simulink model "ASM_Traffic_V2X_Complete_Model_2"  (R2019a)
(part 8 of 36)

  Angle_RL_Wheel[Toe;Camber][deg]/2 -> SignalFilter/624  "<Angle_Camber_RL_Wheel_CoorSys_V[deg]>"
  Angle_RR_Wheel[Toe;Camber][deg]/1 -> SignalFilter/625  "<Angle_Toe_RR_Wheel_CoorSys_V[deg]>"
  Angle_RR_Wheel[Toe;Camber][deg]/2 -> SignalFilter/626  "<Angle_Camber_RR_Wheel_CoorSys_V[deg]>"
  EngineTorques/1 -> SignalFilter/627  "<Const_TimeConst[s]>"
  EngineTorques/2 -> SignalFilter/628  "<Trq_Eff_Engine[Nm]>"
  EngineTorques/3 -> SignalFilter/629  "<Trq_Driver_Des[Nm]>"
  EngineTorques/4 -> SignalFilter/630  "<Trq_Fric_Engine[Nm]>"
  EngineTorques/5 -> SignalFilter/631  "<Trq_Ind_Engine[Nm]>"
  EngineTorques/6 -> SignalFilter/632  "<Trq_FullLoad_Engine[Nm]>"
  FuelConsumption/1 -> SignalFilter/633  "<mdot_Fuel[g|h]>"
  FuelConsumption/2 -> SignalFilter/634  "<b_e[g|kWh]>"
  Efficiency/1 -> SignalFilter/635  "<eta_Eff_Engine[0_1]>"
  Efficiency/2 -> SignalFilter/636  "<eta_Ind_Engine[0_1]>"
  Efficiency/3 -> SignalFilter/637  "<eta_Mechanical_Engine[0_1]>"
  CO2_Emission/1 -> SignalFilter/638  "<CO2_Emission[kg|h]>"
  CO2_Emission/2 -> SignalFilter/639  "<CO2_Emission_Total[kg]>"
  FuelConsumption/5 -> SignalFilter/640  "<Fuel_Consumption[l|h]>"
  FuelConsumption/6 -> SignalFilter/641  "<Fuel_Consumption_Total[l]>"
  ActiveTransmission/1 -> SignalFilter/642  "<Gear[]>"
  ActiveTransmission/2 -> SignalFilter/643  "<omega_In_Trm[rad|s]>"
  ActiveTransmission/3 -> SignalFilter/644  "<omega_Out_Trm[rad|s]>"
  ActiveTransmission/4 -> SignalFilter/645  "<Trq_Out_Trm[Nm]>"
  ActiveTransmission/5 -> SignalFilter/646  "<i_Trm[]>"
  ActiveTransmission/6 -> SignalFilter/647  "<Inertia_Trm[kgm2]>"
  ActiveTransmission/7 -> SignalFilter/648  "<i_unsync_Trm[]>"
  Clutch/1 -> SignalFilter/649  "<Trq_Fric_Clutch[Nm]>"
  Clutch/2 -> SignalFilter/650  "<Trq_TorsionSpring_Clutch[Nm]>"
  Clutch/3 -> SignalFilter/651  "<omega_Out_ClutchPlate[rad|s]>"
  GearBox/1 -> SignalFilter/652  "<i_unsync_Trm[]>"
  GearBox/2 -> SignalFilter/653  "<i_Trm[]>"
  GearBox/3 -> SignalFilter/654  "<Trq_Out_Trm[Nm]>"
  GearBox/4 -> SignalFilter/655  "<omega_In_Trm[rad|s]>"
  GearBox/5 -> SignalFilter/656  "<Inertia_Trm[kgm2]>"
  GearBox/6 -> SignalFilter/657  "<omega_Out_Trm[rad|s]>"
  LockUpClutch/1 -> SignalFilter/658  "<Trq_Fric_Clutch[Nm]>"
  LockUpClutch/2 -> SignalFilter/659  "<Trq_TorsionSpring_Clutch[Nm]>"
  LockUpClutch/3 -> SignalFilter/660  "<omega_Out_ClutchPlate[rad|s]>"
  GearBox1/1 -> SignalFilter/661  "<i_unsync_Trm[]>"
  GearBox1/2 -> SignalFilter/662  "<i_Trm[]>"
  GearBox1/3 -> SignalFilter/663  "<Trq_Out_Trm[Nm]>"
  GearBox1/4 -> SignalFilter/664  "<omega_In_Trm[rad|s]>"
  GearBox1/5 -> SignalFilter/665  "<Inertia_Trm[kgm2]>"
  GearBox1/6 -> SignalFilter/666  "<omega_Out_Trm[rad|s]>"
  TorqueConverter/1 -> SignalFilter/667  "<Trq_Pump[Nm]>"
  TorqueConverter/2 -> SignalFilter/668  "<Trq_Turbine[Nm]>"
  FinalDriveAssembly/1 -> SignalFilter/669  "<i_FinalDrive[]>"
  CentralDifferential/1 -> SignalFilter/670  "<omega_Out_Front_CentralDiff[rad|s]>"
  CentralDifferential/2 -> SignalFilter/671  "<omega_Out_Rear_CentralDiff[rad|s]>"
  CentralDifferential/3 -> SignalFilter/672  "<omega_In_CentralDiff[rad|s]>"
  CentralDifferential/4 -> SignalFilter/673  "<Trq_Lock[Nm]>"
  CentralDifferential/5 -> SignalFilter/674  "<omega_Cage[rad|s]>"
  CentralDifferential/6 -> SignalFilter/675  "<Const_i_MainReductionGear[]>"
  CentralDifferential/7 -> SignalFilter/676  "<Const_TrqDistribution[]>"
  FrontDifferential/1 -> SignalFilter/677  "<omega_Out_Lef_FrontDifferentialt[rad|s]>"
  FrontDifferential/2 -> SignalFilter/678  "<omega_Out_Right_FrontDifferential[rad|s]>"
  FrontDifferential/3 -> SignalFilter/679  "<omega_In_CentralDiff_FrontDifferential[rad|s]>"
  FrontDifferential/4 -> SignalFilter/680  "<Trq_Lock_FrontDifferential[Nm]>"
  FrontDifferential/5 -> SignalFilter/681  "<omega_Cage[rad|s]>"
  FrontDifferential/6 -> SignalFilter/682  "<Const_i_MainReductionGear[]>"
  FrontDifferential/7 -> SignalFilter/683  "<Const_TrqDistribution[]>"
  RearDifferential/1 -> SignalFilter/684  "<omega_Out_Lef_RearDifferentialt[rad|s]>"
  RearDifferential/2 -> SignalFilter/685  "<omega_Out_Right_RearDifferential[rad|s]>"
  RearDifferential/3 -> SignalFilter/686  "<omega_In_CentralDiff_RearDifferential[rad|s]>"
  RearDifferential/4 -> SignalFilter/687  "<Trq_Lock_RearDifferential[Nm]>"
  RearDifferential/5 -> SignalFilter/688  "<omega_Cage[rad|s]>"
  RearDifferential/6 -> SignalFilter/689  "<Const_i_MainReductionGear[]>"
  RearDifferential/7 -> SignalFilter/690  "<Const_TrqDistribution[]>"
  Shaft_TGCL4WD/1 -> SignalFilter/691  "<Trq_TGCL4WD_Shaft[Nm]>"
  Shaft_TGCL4WD/2 -> SignalFilter/692  "<omega_Delta_TGCL4WD_Shaft[rad|s]>"
  Shaft_CF/1 -> SignalFilter/693  "<Trq_CF_Shaft[Nm]>"
  Shaft_CF/2 -> SignalFilter/694  "<omega_Delta_CF_Shaft[rad|s]>"
  Shaft_CR/1 -> SignalFilter/695  "<Trq_CR_Shaft[Nm]>"
  Shaft_CR/2 -> SignalFilter/696  "<omega_Delta_CR_Shaft[rad|s]>"
  TransferGearbox/1 -> SignalFilter/697  "<Trq_In_Transfer_Gearbox[Nm]>"
  TransferGearbox/2 -> SignalFilter/698  "<omega_Out_Transfer_Gearbox[rad|s]>"
  Clutch_4WD/1 -> SignalFilter/699  "<Trq_Lock_Clutch_4WD[Nm]>"
  Clutch_4WD/2 -> SignalFilter/700  "<omega_Clutch_4WD_In[rad|s]>"
  Clutch_4WD/3 -> SignalFilter/701  "<omega_Clutch_4WD_Out[rad|s]>"
  Shaft_FL/1 -> SignalFilter/702  "<Trq_FL_Shaft[Nm]>"
  Shaft_FL/2 -> SignalFilter/703  "<omega_Delta_FL_Shaft[rad|s]>"
  Shaft_FR/1 -> SignalFilter/704  "<Trq_FR_Shaft[Nm]>"
  Shaft_FR/2 -> SignalFilter/705  "<omega_Delta_FR_Shaft[rad|s]>"
  Shaft_RL/1 -> SignalFilter/706  "<Trq_RL_Shaft[Nm]>"
  Shaft_RL/2 -> SignalFilter/707  "<omega_Delta_RL_Shaft[rad|s]>"
  Shaft_RR/1 -> SignalFilter/708  "<Trq_RR_Shaft[Nm]>"
  Shaft_RR/2 -> SignalFilter/709  "<omega_Delta_RR_Shaft[rad|s]>"
  Crankshaft/1 -> SignalFilter/710  "<n_Engine[rad|s]>"
  Crankshaft/2 -> SignalFilter/711  "<n_Engine[rpm]>"
  Crankshaft/3 -> SignalFilter/712  "<Trq_Mass_Mod[Nm]>"
  Crankshaft/4 -> SignalFilter/713  "<Const_Inertia_Engine[kgm2]>"
  Crankshaft/5 -> SignalFilter/714  "<Trq_Eff_Crank[Nm]>"
  Starter/1 -> SignalFilter/715  "<Trq_Starter[Nm]>"
  Starter/2 -> SignalFilter/716  "<Inertia_Starter[kgm2]>"
  TestBench/1 -> SignalFilter/717  "<Trq_TestBench[Nm]>"
  TestBench/2 -> SignalFilter/718  "<Inertia_TestBench[kgm2]>"
  OutputSignals/1 -> SignalFilter/719  "<Pos_AccPedal[%]>"
  OutputSignals/2 -> SignalFilter/720  "<Pos_BrakePedal[%]>"
  OutputSignals/3 -> SignalFilter/721  "<Pos_ClutchPedal[%]>"
  OutputSignals/4 -> SignalFilter/722  "<Gear[]>"
  OutputSignals/5 -> SignalFilter/723  "<t_Preview_vRef[s]>"
  OutputSignals/6 -> SignalFilter/724  "<Angle_SteeringWheel[deg]>"
  AutomaticTrmCtrlSignals/1 -> SignalFilter/725  "<SelectorLever[-3T|-2P|-1R|0N|1D]>"
  AutomaticTrmCtrlSignals/2 -> SignalFilter/726  "<SW_TipTronic[-1Down|0Off|1Up]>"
  StartButtonSignals/1 -> SignalFilter/727  "<Sw_StartButton[0Off|1On]>"
  ParkingBrakeSignals/1 -> SignalFilter/728  "<Sw_ParkingBrake[0Off|1On]>"
  LongCtrl/1 -> SignalFilter/729  "<t_Preview[s]>"
  LongCtrl/2 -> SignalFilter/730  "<Pos_AccPedal[%]>"
  LongCtrl/3 -> SignalFilter/731  "<Pos_BrakePedal[%]>"
  GearShifter/1 -> SignalFilter/732  "<Pos_AccPedal[%]>"
  GearShifter/2 -> SignalFilter/733  "<Pos_BrakePedal[%]>"
  GearShifter/3 -> SignalFilter/734  "<Pos_ClutchPedal[%]>"
  GearShifter/4 -> SignalFilter/735  "<Gear[]>"
  GearShifter/5 -> SignalFilter/736  "<SelectorLever[-3T|-2P|-1R|0N|1D]>"
  ReferenceVelocity/1 -> SignalFilter/737  "<v_Road[km|h]>"
  ReferenceVelocity/2 -> SignalFilter/738  "<s_Preview_vRef[m]>"
  ReferenceVelocity/3 -> SignalFilter/739  "<a_x_Vehicle_Ref[m|s2]>"
  ReferenceVelocity/4 -> SignalFilter/740  "<v_Vehicle_Ref[m|s]>"
  ReferenceVelocity/5 -> SignalFilter/741  "<v_Vehicle_Ref[km|h]>"
  ActiveLateralController/1 -> SignalFilter/742  "<s_Preview_LatCtrl[m]>"
  ActiveLateralController/2 -> SignalFilter/743  "<Angle_SteeringWheel_LatCtrl[deg]>"
  ActiveLateralController/3 -> SignalFilter/744  "<e_Lat[m]>"
  LatCtrl1/1 -> SignalFilter/745  "<s_Preview_Lat[m]>"
  LatCtrl1/2 -> SignalFilter/746  "<Angle_Steering[rad]>"
  LatCtrl1/3 -> SignalFilter/747  "<Angle_SteeringWheel[deg]>"
  LatCtrl2/1 -> SignalFilter/748  "<Angle_SteeringWheel[deg]>"
  LatCtrl2/2 -> SignalFilter/749  "<Angle_Steering[deg]>"
  LatCtrl2/3 -> SignalFilter/750  "<s_Preview_Lat[m]>"
  LatCtrl2/4 -> SignalFilter/751  "<e_Yaw[deg]>"
  LatCtrl2/5 -> SignalFilter/752  "<e_Lat[m]>"
  LatCtrl2/6 -> Reshape_753/1  "<e_Lat_Preview[m]>"
  Reshape_753/1 -> SignalFilter/753
  PositionError/1 -> SignalFilter/754  "<e_Lat[m]>"
  PositionError/2 -> SignalFilter/755  "<e_Lat_Abs[m]>"
  PositionError/3 -> SignalFilter/756  "<e_Lat_Total[m]>"
  Pos_Vehicle_Init_CoorSys_E[x;y;z][m]/1 -> SignalFilter/757  "<Const_Pos_x_Vehicle_Init[m]>"
  Pos_Vehicle_Init_CoorSys_E[x;y;z][m]/2 -> SignalFilter/758  "<Const_Pos_y_Vehicle_Init[m]>"
  Pos_Vehicle_Init_CoorSys_E[x;y;z][m]/3 -> SignalFilter/759  "<Const_Pos_z_Vehicle_Init[m]>"
  Angle_Vehicle_Init_CoorSys_E[x;y;z][rad]/1 -> SignalFilter/760  "<Angle_Roll_Vehicle_Init[rad]>"
  Angle_Vehicle_Init_CoorSys_E[x;y;z][rad]/2 -> SignalFilter/761  "<Angle_Pitch_Vehicle_Init[rad]>"
  Angle_Vehicle_Init_CoorSys_E[x;y;z][rad]/3 -> SignalFilter/762  "<Angle_Yaw_Vehicle_Init[rad]>"
  Road_ASMVeh/1 -> SignalFilter/763  "<s_Veh_Road[m]>"
  Road_ASMVeh/2 -> SignalFilter/764  "<s_Total_Veh_Road[m]>"
  Road_ASMVeh/3 -> SignalFilter/765  "<d_Total_Veh_Road[m]>"
  Road_ASMVeh/4 -> SignalFilter/766  "<s_Veh_Road_Trj[m]>"
  Road_ASMVeh/5 -> SignalFilter/767  "<LaneIdx_Total_Veh_Road[]>"
  Road_ASMVeh/6 -> SignalFilter/768  "<Curv_Veh_Road[1|m]>"
  Road_ASMVeh/7 -> SignalFilter/769  "<Pos_x_Ref_Veh_Road[m]>"
  Road_ASMVeh/8 -> SignalFilter/770  "<Pos_y_Ref_Veh_Road[m]>"
  Road_ASMVeh/9 -> SignalFilter/771  "<Angle_Yaw_Veh_Road[deg]>"
  Road_ASMVeh/10 -> SignalFilter/772  "<Slope_Veh_Road[%]>"
  Road_ASMVeh/11 -> Reshape_773/1  "<v_Wind_Coor_Sys_E[x;y;z][m|s]>"
  Reshape_773/1 -> SignalFilter/773
  Road_ASMVeh/12 -> SignalFilter/774  "<Slope_Lateral_Veh_Road[deg]>"
  Road_ContactPoints/1 -> Reshape_775/1  "<Pos_z_CP[:][m]>"
  Reshape_775/1 -> SignalFilter/775
  Road_ContactPoints/2 -> Reshape_776/1  "<Fric_Coeff_CP[:][]>"
  Reshape_776/1 -> SignalFilter/776
  Road_ContactPoints/3 -> Reshape_777/1  "<UnitVec_z_CP[:][x;y;z]>"
  Reshape_777/1 -> SignalFilter/777
  Road_ContactPoints/4 -> Reshape_778/1  "<Sw_Tire_Parameter_Set_CP[:][1|2|3|4]>"
  Reshape_778/1 -> SignalFilter/778
  Road_Preview/1 -> Reshape_779/1  "<Pos_x_Preview_Road[m]>"
  Reshape_779/1 -> SignalFilter/779
  Road_Preview/2 -> Reshape_780/1  "<Pos_y_Preview_Road[m]>"
  Reshape_780/1 -> SignalFilter/780
  Road_Preview/3 -> Reshape_781/1  "<Curv_Preview_Road[1|m]>"
  Reshape_781/1 -> SignalFilter/781
  Road_Preview/4 -> Reshape_782/1  "<Speed_Limit_Preview_Road[km|h]>"
  Reshape_782/1 -> SignalFilter/782
  Road_Preview/5 -> Reshape_783/1  "<Pos_z_Preview_Road[m]>"
  Reshape_783/1 -> SignalFilter/783
  Road_Preview/6 -> Reshape_784/1  "<Roll_Preview_Road[deg]>"
  Reshape_784/1 -> SignalFilter/784
  Road_Preview/7 -> Reshape_785/1  "<Pitch_Preview_Road[deg]>"
  Reshape_785/1 -> SignalFilter/785
  Road_Preview/8 -> Reshape_786/1  "<x_Preview_DriverCurv[m]>"
  Reshape_786/1 -> SignalFilter/786
  Road_Preview/9 -> Reshape_787/1  "<y_Preview_DriverCurv[m]>"
  Reshape_787/1 -> SignalFilter/787
  Road_Info/1 -> SignalFilter/788  "<RoadState[]>"
  Road_Info/2 -> SignalFilter/789  "<RouteLength_Veh[m]>"
  Road_Info/3 -> SignalFilter/790  "<Flag_RouteClosed_Veh[0|1]>"
  Dist_Response_Maneuver/1 -> SignalFilter/791  "<Distance_xy[m]>"
  Dist_Response_Maneuver/2 -> SignalFilter/792  "<Distance_z[m]>"
  Road_Info/5 -> SignalFilter/793  "<Speed_Limit_Veh[km|h]>"
  Road_Info/6 -> SignalFilter/794  "<Network_Item_Type_Veh[]>"
  Road_Info/7 -> SignalFilter/795  "<Network_Item_Id_Veh[]>"
  Road_Info/8 -> SignalFilter/796  "<RoadSegment_Veh[]>"
  Road_Info/9 -> SignalFilter/797  "<LaneSection_Veh[]>"
  Road_Info/10 -> SignalFilter/798  "<RoadWidth_Veh[m]>"
  Road_Info/11 -> SignalFilter/799  "<Network_Load_Idx[]>"
  Road_Info/12 -> SignalFilter/800  "<d_Veh_Ref_Line[m]>"
  Road_Info/13 -> SignalFilter/801  "<Dist_Border_Left[m]>"
  Road_Info/14 -> SignalFilter/802  "<Dist_Border_Right[m]>"
  Road_TrafficFellows/1 -> Reshape_803/1  "<Pos_x_Fellows_Road[m]>"
  Reshape_803/1 -> SignalFilter/803
  Road_TrafficFellows/2 -> Reshape_804/1  "<Pos_y_Fellows_Road[m]>"
  Reshape_804/1 -> SignalFilter/804
  Road_TrafficFellows/3 -> Reshape_805/1  "<Pos_z_Fellows_Road[m]>"
  Reshape_805/1 -> SignalFilter/805
  Road_TrafficFellows/4 -> Reshape_806/1  "<Angle_Yaw_Fellows_Road[deg]>"
  Reshape_806/1 -> SignalFilter/806
  Road_TrafficFellows/5 -> Reshape_807/1  "<Angle_Pitch_Fellows_Road[deg]>"
  Reshape_807/1 -> SignalFilter/807
  Road_TrafficFellows/6 -> Reshape_808/1  "<Angle_Roll_Fellows_Road[deg]>"
  Reshape_808/1 -> SignalFilter/808
  Road_TrafficFellows/7 -> Reshape_809/1  "<Curv_Fellows_Road[1|m]>"
  Reshape_809/1 -> SignalFilter/809
  Road_TrafficFellows/8 -> Reshape_810/1  "<d_Total_Fellows_Road[m]>"
  Reshape_810/1 -> SignalFilter/810
  Road_TrafficFellows/9 -> Reshape_811/1  "<LaneIdx_Total_Fellows_Road[]>"
  Reshape_811/1 -> SignalFilter/811
  Road_TrafficFellows/10 -> Reshape_812/1  "<RoadSegment_Fellows[]>"
  Reshape_812/1 -> SignalFilter/812
  Road_TrafficFellows/11 -> Reshape_813/1  "<LaneSection_Fellows[]>"
  Reshape_813/1 -> SignalFilter/813
  Road_TrafficFellows/12 -> Reshape_814/1  "<Speed_Limit_Fellows[]>"
  Reshape_814/1 -> SignalFilter/814
  Road_TrafficFellows/13 -> Reshape_815/1  "<Network_Item_Type_Fellows[]>"
  Reshape_815/1 -> SignalFilter/815
  Road_TrafficFellows/14 -> Reshape_816/1  "<Network_Item_Id_Fellows[]>"
  Reshape_816/1 -> SignalFilter/816
  Road_TrafficFellows/15 -> Reshape_817/1  "<d_Fellows_RefLine[m]>"
  Reshape_817/1 -> SignalFilter/817
  Road_TrafficFellows/16 -> Reshape_818/1  "<RouteLength_Fellows[m]>"
  Reshape_818/1 -> SignalFilter/818
  Road_TrafficFellows/17 -> Reshape_819/1  "<Flag_RouteClosed_Fellows[0|1]>"
  Reshape_819/1 -> SignalFilter/819
  Dist_Response_Traffic/1 -> Reshape_820/1  "<Distance_xy[m]>"
  Reshape_820/1 -> SignalFilter/820
  Dist_Response_Traffic/2 -> Reshape_821/1  "<Distance_z[m]>"
  Reshape_821/1 -> SignalFilter/821
  Road_TrafficFellows/19 -> Reshape_822/1  "<Angle_Yaw_Fellows_RoadRefline[deg]>"
  Reshape_822/1 -> SignalFilter/822
  UserSignals/1 -> SignalFilter/823  "<User1[]>"
  UserSignals/2 -> SignalFilter/824  "<User2[]>"
  UserSignals/3 -> SignalFilter/825  "<User3[]>"
  UserSignals/4 -> SignalFilter/826  "<User4[]>"
  UserSignals/5 -> SignalFilter/827  "<User5[]>"
  UserSignals/6 -> SignalFilter/828  "<User6[]>"
  UserSignals/7 -> SignalFilter/829  "<User7[]>"
  UserSignals/8 -> SignalFilter/830  "<User8[]>"
  UserSignals/9 -> SignalFilter/831  "<User9[]>"
  UserSignals/10 -> SignalFilter/832  "<User10[]>"
  UserSignals_Customized/1 -> SignalFilter/833  "<GPS_Method[]>"
  UserSignals_Customized/2 -> SignalFilter/834  "<Const_Offset_Lat[deg]>"
  UserSignals_Customized/3 -> SignalFilter/835  "<Const_Offset_Long[deg]>"
  Pos_Vehicle_GPS[Long;Lat][deg]/1 -> SignalFilter/836  "<Longitude[deg]>"
  Pos_Vehicle_GPS[Long;Lat][deg]/2 -> SignalFilter/837  "<Latitude[deg]>"
  Ambient/1 -> SignalFilter/838  "<T_Ambient[degC]>"
  Ambient/2 -> SignalFilter/839  "<p_Ambient[Pa]>"
  Parameters/1 -> Reshape_840/1  "<Enable_Evaluation[0|1]>"
  Reshape_840/1 -> SignalFilter/840
  Parameters/2 -> Reshape_841/1  "<Evaluation_Distance[m]>"
  Reshape_841/1 -> SignalFilter/841
  Parameters/3 -> SignalFilter/842  "<Border_Mode[0Center|1Inner|2Outer]>"
  Parameters/4 -> SignalFilter/843  "<Enable_Junction_Evaluation[0|1]>"
  Parameters/5 -> Reshape_844/1  "<Num_Lanes[Left;Right]>"
  Reshape_844/1 -> SignalFilter/844
  Parameters/6 -> Reshape_845/1  "<Enable_MeasPoint[0|1]>"
  Reshape_845/1 -> SignalFilter/845
  Parameters/7 -> Reshape_846/1  "<MeasPoint_1_CoorSysV[x;y][m]>"
  Reshape_846/1 -> SignalFilter/846
  Parameters/8 -> Reshape_847/1  "<MeasPoint_2_CoorSysV[x;y][m]>"
  Reshape_847/1 -> SignalFilter/847
  Parameters/9 -> Reshape_848/1  "<MeasPoint_3_CoorSysV[x;y][m]>"
  Reshape_848/1 -> SignalFilter/848
  Parameters/10 -> Reshape_849/1  "<MeasPoint_4_CoorSysV[x;y][m]>"
  Reshape_849/1 -> SignalFilter/849
  Parameters/11 -> Reshape_850/1  "<MeasPoint_1_CoorSysE[x;y][m]>"
  Reshape_850/1 -> SignalFilter/850
  Parameters/12 -> Reshape_851/1  "<MeasPoint_2_CoorSysE[x;y][m]>"
  Reshape_851/1 -> SignalFilter/851
  Parameters/13 -> Reshape_852/1  "<MeasPoint_3_CoorSysE[x;y][m]>"
  Reshape_852/1 -> SignalFilter/852
  Parameters/14 -> Reshape_853/1  "<MeasPoint_4_CoorSysE[x;y][m]>"
  Reshape_853/1 -> SignalFilter/853
  SFunction_Info/1 -> SignalFilter/854  "<Sfcn_State[0|1]>"
  SFunction_Info/2 -> SignalFilter/855  "<Input_Data_Valid[0|1]>"
  SFunction_Info/3 -> DataTypeConversion_856/1  "<Data_Valid[0|1]>"
  DataTypeConversion_856/1 -> SignalFilter/856
  Network_Item/1 -> SignalFilter/857  "<Network_Item_ID[]>"
  Network_Item/2 -> SignalFilter/858  "<Network_Item_Type[]>"
  Network_Item/3 -> SignalFilter/859  "<Network_Item_Type_Absolute[]>"
  Network_Item/4 -> SignalFilter/860  "<Preferred_Lane_Direct[]>"
  Network_Item/5 -> SignalFilter/861  "<Preferred_Lane_Oncoming[]>"
  Common/1 -> SignalFilter/862  "<LaneID_PrefLane[]>"
  Common/2 -> SignalFilter/863  "<LaneID_Absolute[]>"
  Common/3 -> SignalFilter/864  "<LaneDirection_Absolute[]>"
  Common/4 -> SignalFilter/865  "<LaneDirection_Relative[]>"
  Common/5 -> SignalFilter/866  "<LaneWidth[m]>"
  Common/6 -> SignalFilter/867  "<LaneCurvature[1|m]>"
  Common/7 -> SignalFilter/868  "<Curvature[1|m]>"
  LeftSide/1 -> Reshape_869/1  "<Pos_Left[x;y;z][m]>"
  Reshape_869/1 -> SignalFilter/869
  LeftSide/2 -> SignalFilter/870  "<Yaw_Angle_Left[deg]>"
  LeftSide/3 -> SignalFilter/871  "<Yaw_Angle_RelVehicle_Left[deg]>"
  LeftSide/4 -> SignalFilter/872  "<Curvature_Left[1|m]>"
  LeftSide/5 -> SignalFilter/873  "<MarkerType_Left[]>"
  LeftSide/6 -> SignalFilter/874  "<MarkerWidth_Left[m]>"
  LeftSide/7 -> SignalFilter/875  "<MarkerColor_Left[]>"
  LeftSide/8 -> SignalFilter/876  "<LineID_1_Left[]>"
  LeftSide/9 -> SignalFilter/877  "<LineID_2_Left[]>"
  LeftSide/10 -> SignalFilter/878  "<Distance_Marker_Left[m]>"
  RightSide/1 -> Reshape_879/1  "<Pos_Right[x;y;z][m]>"
  Reshape_879/1 -> SignalFilter/879
  RightSide/2 -> SignalFilter/880  "<Yaw_Angle_Right[deg]>"
  RightSide/3 -> SignalFilter/881  "<Yaw_Angle_RelVehicle_Right[deg]>"
  RightSide/4 -> SignalFilter/882  "<Curvature_Right[1|m]>"
  RightSide/5 -> SignalFilter/883  "<MarkerType_Right[]>"
  RightSide/6 -> SignalFilter/884  "<MarkerWidth_Right[m]>"
  RightSide/7 -> SignalFilter/885  "<MarkerColor_Right[]>"
  RightSide/8 -> SignalFilter/886  "<LineID_1_Right[]>"
  RightSide/9 -> SignalFilter/887  "<LineID_2_Right[]>"
  RightSide/10 -> SignalFilter/888  "<Distance_Marker_Right[m]>"
  Lanes_Left/1 -> Reshape_889/1  "<LaneID_PrefLane[]>"
  Reshape_889/1 -> SignalFilter/889
  Lanes_Left/2 -> Reshape_890/1  "<LaneID_Absolute[]>"
  Reshape_890/1 -> SignalFilter/890
  Lanes_Left/3 -> Reshape_891/1  "<LaneDirection_Absolute[]>"
  Reshape_891/1 -> SignalFilter/891
  Lanes_Left/4 -> Reshape_892/1  "<LaneDirection_Relative[]>"
  Reshape_892/1 -> SignalFilter/892
  Lanes_Left/5 -> Reshape_893/1  "<LaneWidth[m]>"
  Reshape_893/1 -> SignalFilter/893
  Lanes_Left/6 -> Reshape_894/1  "<LaneCurvature[1|m]>"
  Reshape_894/1 -> SignalFilter/894
  Lanes_Left/7 -> Reshape_895/1  "<Pos_Left[x;y;z][m]>"
  Reshape_895/1 -> SignalFilter/895
  Lanes_Left/8 -> Reshape_896/1  "<Yaw_Angle_Left[deg]>"
  Reshape_896/1 -> SignalFilter/896
  Lanes_Left/9 -> Reshape_897/1  "<Yaw_Angle_RelVehicle_Left[deg]>"
  Reshape_897/1 -> SignalFilter/897
  Lanes_Left/10 -> Reshape_898/1  "<Curvature_Left[1|m]>"
  Reshape_898/1 -> SignalFilter/898
  Lanes_Left/11 -> Reshape_899/1  "<MarkerType_Left[]>"
  Reshape_899/1 -> SignalFilter/899
  Lanes_Left/12 -> Reshape_900/1  "<MarkerWidth_Left[m]>"
  Reshape_900/1 -> SignalFilter/900
  Lanes_Left/13 -> Reshape_901/1  "<MarkerColor_Left[]>"
  Reshape_901/1 -> SignalFilter/901
  Lanes_Left/14 -> Reshape_902/1  "<LineID_1_Left[]>"
  Reshape_902/1 -> SignalFilter/902
  Lanes_Left/15 -> Reshape_903/1  "<LineID_2_Left[]>"
  Reshape_903/1 -> SignalFilter/903
  Lanes_Left/16 -> Reshape_904/1  "<Distance_Marker_Left[m]>"
  Reshape_904/1 -> SignalFilter/904
  Lanes_Left/17 -> Reshape_905/1  "<Pos_Right[x;y;z][m]>"
  Reshape_905/1 -> SignalFilter/905
  Lanes_Left/18 -> Reshape_906/1  "<Yaw_Angle_Right[deg]>"
  Reshape_906/1 -> SignalFilter/906
  Lanes_Left/19 -> Reshape_907/1  "<Yaw_Angle_RelVehicle_Right[deg]>"
  Reshape_907/1 -> SignalFilter/907
  Lanes_Left/20 -> Reshape_908/1  "<Curvature_Right[1|m]>"
  Reshape_908/1 -> SignalFilter/908
  Lanes_Left/21 -> Reshape_909/1  "<MarkerType_Right[]>"
  Reshape_909/1 -> SignalFilter/909
  Lanes_Left/22 -> Reshape_910/1  "<MarkerWidth_Right[m]>"
  Reshape_910/1 -> SignalFilter/910
  Lanes_Left/23 -> Reshape_911/1  "<MarkerColor_Right[]>"
  Reshape_911/1 -> SignalFilter/911
  Lanes_Left/24 -> Reshape_912/1  "<LineID_1_Right[]>"
  Reshape_912/1 -> SignalFilter/912
  Lanes_Left/25 -> Reshape_913/1  "<LineID_2_Right[]>"
  Reshape_913/1 -> SignalFilter/913
  Lanes_Left/26 -> Reshape_914/1  "<Distance_Marker_Right[m]>"
  Reshape_914/1 -> SignalFilter/914
  Lanes_Right/1 -> Reshape_915/1  "<LaneID_PrefLane[]>"
  Reshape_915/1 -> SignalFilter/915
  Lanes_Right/2 -> Reshape_916/1  "<LaneID_Absolute[]>"
  Reshape_916/1 -> SignalFilter/916
  Lanes_Right/3 -> Reshape_917/1  "<LaneDirection_Absolute[]>"
  Reshape_917/1 -> SignalFilter/917
  Lanes_Right/4 -> Reshape_918/1  "<LaneDirection_Relative[]>"
  Reshape_918/1 -> SignalFilter/918
  Lanes_Right/5 -> Reshape_919/1  "<LaneWidth[m]>"
  Reshape_919/1 -> SignalFilter/919
  Lanes_Right/6 -> Reshape_920/1  "<LaneCurvature[1|m]>"
  Reshape_920/1 -> SignalFilter/920
  Lanes_Right/7 -> Reshape_921/1  "<Pos_Left[x;y;z][m]>"
  Reshape_921/1 -> SignalFilter/921
  Lanes_Right/8 -> Reshape_922/1  "<Yaw_Angle_Left[deg]>"
  Reshape_922/1 -> SignalFilter/922
  Lanes_Right/9 -> Reshape_923/1  "<Yaw_Angle_RelVehicle_Left[deg]>"
  Reshape_923/1 -> SignalFilter/923
  Lanes_Right/10 -> Reshape_924/1  "<Curvature_Left[1|m]>"
  Reshape_924/1 -> SignalFilter/924
  Lanes_Right/11 -> Reshape_925/1  "<MarkerType_Left[]>"
  Reshape_925/1 -> SignalFilter/925
  Lanes_Right/12 -> Reshape_926/1  "<MarkerWidth_Left[m]>"
  Reshape_926/1 -> SignalFilter/926
  Lanes_Right/13 -> Reshape_927/1  "<MarkerColor_Left[]>"
  Reshape_927/1 -> SignalFilter/927
  Lanes_Right/14 -> Reshape_928/1  "<LineID_1_Left[]>"
  Reshape_928/1 -> SignalFilter/928
  Lanes_Right/15 -> Reshape_929/1  "<LineID_2_Left[]>"
  Reshape_929/1 -> SignalFilter/929
  Lanes_Right/16 -> Reshape_930/1  "<Distance_Marker_Left[m]>"
  Reshape_930/1 -> SignalFilter/930
  Lanes_Right/17 -> Reshape_931/1  "<Pos_Right[x;y;z][m]>"
  Reshape_931/1 -> SignalFilter/931
  Lanes_Right/18 -> Reshape_932/1  "<Yaw_Angle_Right[deg]>"
  Reshape_932/1 -> SignalFilter/932
  Lanes_Right/19 -> Reshape_933/1  "<Yaw_Angle_RelVehicle_Right[deg]>"
  Reshape_933/1 -> SignalFilter/933
  Lanes_Right/20 -> Reshape_934/1  "<Curvature_Right[1|m]>"
  Reshape_934/1 -> SignalFilter/934
  Lanes_Right/21 -> Reshape_935/1  "<MarkerType_Right[]>"
  Reshape_935/1 -> SignalFilter/935
  Lanes_Right/22 -> Reshape_936/1  "<MarkerWidth_Right[m]>"
  Reshape_936/1 -> SignalFilter/936
  Lanes_Right/23 -> Reshape_937/1  "<MarkerColor_Right[]>"
  Reshape_937/1 -> SignalFilter/937
  Lanes_Right/24 -> Reshape_938/1  "<LineID_1_Right[]>"
  Reshape_938/1 -> SignalFilter/938
  Lanes_Right/25 -> Reshape_939/1  "<LineID_2_Right[]>"
  Reshape_939/1 -> SignalFilter/939
  Lanes_Right/26 -> Reshape_940/1  "<Distance_Marker_Right[m]>"
  Reshape_940/1 -> SignalFilter/940
  Measurement_Points/1 -> Reshape_941/1  "<Distance_MeasPnt_Marker_Left[m]>"
  Reshape_941/1 -> SignalFilter/941
  Measurement_Points/2 -> Reshape_942/1  "<Distance_MeasPnt_Marker_Right[m]>"
  Reshape_942/1 -> SignalFilter/942
  Measurement_Points/3 -> Reshape_943/1  "<Velocity_MeasPnt_Marker_Left[m|s]>"
  Reshape_943/1 -> SignalFilter/943
  Measurement_Points/4 -> Reshape_944/1  "<Velocity_MeasPnt_Marker_Right[m|s]>"
  Reshape_944/1 -> SignalFilter/944
  MdlControl/1 -> SignalFilter/945  "<Reset_VehicleStates[0|1]>"
  MdlControl/2 -> SignalFilter/946  "<RoadControl[]>"
  MdlControl/3 -> SignalFilter/947  "<Get_VehPos_Trigger[]>"
  MdlControl/4 -> SignalFilter/948  "<Keep_VehiclePosition[0|1]>"
  InitialVehStates/1 -> SignalFilter/949  "<s_Vehicle_Init[m]>"
  InitialVehStates/2 -> SignalFilter/950  "<d_Vehicle_Init[m]>"
  InitialVehStates/3 -> SignalFilter/951  "<LaneIdx_Vehicle_Init[]>"
  InitialVehStates/4 -> SignalFilter/952  "<Pos_z_Vehicle_Rel_Init[m]>"
  InitialVehStates/5 -> SignalFilter/953  "<Angle_Yaw_Vehicle_Rel_Init[deg]>"
  InitialVehStates/6 -> SignalFilter/954  "<v_Vehicle_Init[km|h]>"
  InitialVehStates/7 -> SignalFilter/955  "<Route_Id_Init[]>"
  InitialVehStates/8 -> SignalFilter/956  "<Route_Direction_Init[]>"
  ModeSignals/1 -> SignalFilter/957  "<AccBr_Mode[1Stim|2Driver]>"
  ModeSignals/2 -> SignalFilter/958  "<GearClutch_Mode[1Stim|2Driver|3OpenClutch|4RefGear]>"
  ModeSignals/3 -> SignalFilter/959  "<Steer_Mode[1Stim|2Driver|3Fix]>"
  ModeSignals/4 -> SignalFilter/960  "<Road_Mode[1NoRoad|2Straight|3Circle|4Road]>"
  ModeSignals/5 -> SignalFilter/961  "<LatDriver[1LatCtrl1|2LatCtrl2]>"
  ModeSignals/6 -> SignalFilter/962  "<LatCtrl_Mode[1Pos|2Yaw]>"
  ModeSignals/7 -> SignalFilter/963  "<AdaptVelocityToRoad_Mode[1Off|2On]>"
  ModeSignals/8 -> SignalFilter/964  "<ForceToRoad_Mode[1Off|2On]>"
  ModeSignals/9 -> SignalFilter/965  "<SelectorLever_Mode[1Stim|2Driver]>"
  ModeSignals/10 -> SignalFilter/966  "<CurvatureCalculation_Mode[1Road|2Driver]>"
  RefSignals/1 -> SignalFilter/967  "<Pos_AccPedal_Maneuver[%]>"
  RefSignals/2 -> SignalFilter/968  "<Pos_BrakePedal_Maneuver[%]>"
  RefSignals/3 -> SignalFilter/969  "<Pos_ClutchPedal_Maneuver[%]>"
  RefSignals/4 -> SignalFilter/970  "<Gear_Maneuver[]>"
  RefSignals/5 -> SignalFilter/971  "<Angle_SteeringWheel_Maneuver[deg]>"
  RefSignals/6 -> SignalFilter/972  "<v_Vehicle_Ref_Maneuver[m|s]>"
  RefSignals/7 -> SignalFilter/973  "<d_Maneuver[m]>"
  RefSignals/8 -> SignalFilter/974  "<LaneIdx_Maneuver[]>"
  RefSignals/9 -> Reshape_975/1  "<Dist_Def_Maneuver[]>"
  Reshape_975/1 -> SignalFilter/975
  RefSignals/10 -> SignalFilter/976  "<v_Vehicle_Ref_Preview_Maneuver[m|s]>"
  RefSignals/11 -> SignalFilter/977  "<v_Vehicle_Ref_Preview_State[0Invalid|1CurrentSeg|2NextSeg]>"
  RefSignals/12 -> SignalFilter/978  "<Sw_SteeringMode_Maneuver[1Angle|2Trq]>"
  RefSignals/13 -> SignalFilter/979  "<Trq_Steering_Maneuver[Nm]>"
  RefSignals/14 -> SignalFilter/980  "<SelectorLever_Maneuver[]>"
  RefSignals/15 -> Reshape_981/1  "<Dist_Def_Refline_Maneuver[]>"
  Reshape_981/1 -> SignalFilter/981
  Parameters1/1 -> SignalFilter/982  "<a_x_Max[m|s2]>"
  Parameters1/2 -> SignalFilter/983  "<a_x_Brake_Threshold[m|s2]>"
  Parameters1/3 -> SignalFilter/984  "<a_y_Max[m|s2]>"
  Parameters1/4 -> SignalFilter/985  "<Curv_Road_Circle[1|m]>"
  Parameters1/5 -> SignalFilter/986  "<Gear_Max[]>"
  Parameters1/6 -> SignalFilter/987  "<Width_Deadzone_LatCtrl[m]>"
  Parameters1/7 -> SignalFilter/988  "<v_Lat[m|s]>"
  Parameters1/8 -> SignalFilter/989  "<Object_Type_ID[]>"
  UserSignals1/1 -> SignalFilter/990  "<User1[]>"
  UserSignals1/2 -> SignalFilter/991  "<User2[]>"
  UserSignals1/3 -> SignalFilter/992  "<User3[]>"
  UserSignals1/4 -> SignalFilter/993  "<User4[]>"
  UserSignals1/5 -> SignalFilter/994  "<User5[]>"
  UserSignals1/6 -> SignalFilter/995  "<User6[]>"
  UserSignals1/7 -> SignalFilter/996  "<User7[]>"
  UserSignals1/8 -> SignalFilter/997  "<User8[]>"
  UserSignals1/9 -> SignalFilter/998  "<User9[]>"
  UserSignals1/10 -> SignalFilter/999  "<User10[]>"
  UserSignals1/11 -> SignalFilter/1000  "<User11[]>"
  UserSignals1/12 -> SignalFilter/1001  "<User12[]>"
  UserSignals1/13 -> SignalFilter/1002  "<User13[]>"
  UserSignals1/14 -> SignalFilter/1003  "<User14[]>"
  UserSignals1/15 -> SignalFilter/1004  "<User15[]>"
  UserSignals1/16 -> SignalFilter/1005  "<User16[]>"
  UserSignals1/17 -> SignalFilter/1006  "<User17[]>"
  UserSignals1/18 -> SignalFilter/1007  "<User18[]>"
  UserSignals1/19 -> SignalFilter/1008  "<User19[]>"
  UserSignals1/20 -> SignalFilter/1009  "<User20[]>"
  UserSignals1/21 -> SignalFilter/1010  "<User21[]>"
  UserSignals1/22 -> SignalFilter/1011  "<User22[]>"
  UserSignals1/23 -> SignalFilter/1012  "<User23[]>"
  UserSignals1/24 -> SignalFilter/1013  "<User24[]>"
  UserSignals1/25 -> SignalFilter/1014  "<User25[]>"
  UserSignals1/26 -> SignalFilter/1015  "<User26[]>"
  UserSignals1/27 -> SignalFilter/1016  "<User27[]>"
  UserSignals1/28 -> SignalFilter/1017  "<User28[]>"
  UserSignals1/29 -> SignalFilter/1018  "<User29[]>"
  UserSignals1/30 -> SignalFilter/1019  "<User30[]>"
  Info/1 -> SignalFilter/1020  "<CurrentSegment[]>"
  Info/2 -> SignalFilter/1021  "<t_local[s]>"
  Info/3 -> SignalFilter/1022  "<s_local[m]>"
  Info/4 -> SignalFilter/1023  "<ManeuverTime[s]>"
  Info/5 -> SignalFilter/1024  "<ManeuverState[]>"
  Info/6 -> SignalFilter/1025  "<ErrorFlag[]>"
  Info/7 -> SignalFilter/1026  "<CurrentSequence[]>"
  UserSignals_Customized1/1 -> SignalFilter/1027  "<ExternalSegmentEnd_Mode[]>"
  UserSignals_Customized1/2 -> SignalFilter/1028  "<ExternalSegmentEnd_Value[]>"
  UserSignals_Customized1/3 -> SignalFilter/1029  "<ASM_Vehicle_TurnLights[]>"
  UserSignals_Customized1/4 -> SignalFilter/1030  "<ECU_Commands[]>"
  UserSignals_Customized1/5 -> SignalFilter/1031  "<Mnv_DataStream_5[]>"
  UserSignals_Customized1/6 -> SignalFilter/1032  "<Mnv_DataStream_6[]>"
  UserSignals_Customized1/7 -> SignalFilter/1033  "<Mnv_DataStream_7[]>"
  UserSignals_Customized1/8 -> SignalFilter/1034  "<Mnv_DataStream_8[]>"
  FellowMovement1/1 -> Reshape_1035/1  "<d_Total_Fellows[m]>"
  Reshape_1035/1 -> SignalFilter/1035
  FellowMovement1/2 -> Reshape_1036/1  "<LaneIdx_Total_Fellows[]>"
  Reshape_1036/1 -> SignalFilter/1036
  FellowMovement1/3 -> Reshape_1037/1  "<s_Fellows[m]>"
  Reshape_1037/1 -> SignalFilter/1037
  FellowMovement1/4 -> Reshape_1038/1  "<v_Fellows[km|h]>"
  Reshape_1038/1 -> SignalFilter/1038
  Pos_Fellows_MainPnt_CoorSys_E[x;y;z][m]/1 -> Reshape_1039/1  "<Pos_x_Fellows[m]>"
  Reshape_1039/1 -> SignalFilter/1039
  Pos_Fellows_MainPnt_CoorSys_E[x;y;z][m]/2 -> Reshape_1040/1  "<Pos_y_Fellows[m]>"
  Reshape_1040/1 -> SignalFilter/1040
  Pos_Fellows_MainPnt_CoorSys_E[x;y;z][m]/3 -> Reshape_1041/1  "<Pos_z_Fellows[m]>"
  Reshape_1041/1 -> SignalFilter/1041
  Angle_Fellows[x;y;z][deg]/1 -> Reshape_1042/1  "<Angle_Roll_Fellows[deg]>"
  Reshape_1042/1 -> SignalFilter/1042
  Angle_Fellows[x;y;z][deg]/2 -> Reshape_1043/1  "<Angle_Pitch_Fellows[deg]>"
  Reshape_1043/1 -> SignalFilter/1043
  Angle_Fellows[x;y;z][deg]/3 -> Reshape_1044/1  "<Angle_Yaw_Fellows[deg]>"
  Reshape_1044/1 -> SignalFilter/1044
  Angle_Fellows[x;y;z][deg]/4 -> Reshape_1045/1  "<Angle_Wheel_Fellows[deg]>"
  Reshape_1045/1 -> SignalFilter/1045
  FellowPositions/3 -> Reshape_1046/1  "<Angle_Wheel_Fellows[deg]>"
  Reshape_1046/1 -> SignalFilter/1046
  FellowVelocities/1 -> Reshape_1047/1  "<v_Fellows[x;y;z][km|h]>"
  Reshape_1047/1 -> SignalFilter/1047
  FellowVelocities/2 -> Reshape_1048/1  "<w_Fellows[x;y;z][deg|s]>"
  Reshape_1048/1 -> SignalFilter/1048
  TrafficScheduler/1 -> Reshape_1049/1  "<s_Fellows_Ref_Scheduler[m]>"
  Reshape_1049/1 -> SignalFilter/1049
  TrafficScheduler/2 -> Reshape_1050/1  "<v_Fellows_Ref_Scheduler[km|h]>"
  Reshape_1050/1 -> SignalFilter/1050
  TrafficScheduler/3 -> Reshape_1051/1  "<Angle_Yaw_Fellows_Ref_Scheduler[deg]>"
  Reshape_1051/1 -> SignalFilter/1051
  TrafficScheduler/4 -> Reshape_1052/1  "<d_Fellows_Ref_Scheduler[m]>"
  Reshape_1052/1 -> SignalFilter/1052
  TrafficScheduler/5 -> Reshape_1053/1  "<LaneIdx_Fellows_Ref_Scheduler[]>"
  Reshape_1053/1 -> SignalFilter/1053
  TrafficScheduler/6 -> Reshape_1054/1  "<ForceToRoad_Fellows_Ref_Scheduler[0|1]>"
  Reshape_1054/1 -> SignalFilter/1054
  TrafficScheduler/7 -> Reshape_1055/1  "<v_Lat_Fellows_Ref_Scheduler[m|s]>"
  Reshape_1055/1 -> SignalFilter/1055
  TrafficScheduler/8 -> Reshape_1056/1  "<Flag_FellowsUsed[0|1]>"
  Reshape_1056/1 -> SignalFilter/1056
  TrafficScheduler/9 -> Reshape_1057/1  "<Direction_Fellows_Ref_Scheduler[-1|1]>"
  Reshape_1057/1 -> SignalFilter/1057
  TrafficScheduler/10 -> Reshape_1058/1  "<Flag_FellowsMode[0vel|1pos]>"
  Reshape_1058/1 -> SignalFilter/1058
  TrafficScheduler/11 -> Reshape_1059/1  "<Dist_Def_Trf[]>"
  Reshape_1059/1 -> SignalFilter/1059
  TrafficScheduler/12 -> Reshape_1060/1  "<Route_Id_Fellows_Ref_Scheduler[]>"
  Reshape_1060/1 -> SignalFilter/1060
  TrafficScheduler/13 -> Reshape_1061/1  "<UserSignals[]>"
  Reshape_1061/1 -> SignalFilter/1061
  TrafficScheduler/14 -> Reshape_1062/1  "<UserSignals_Fellows[]>"
  Reshape_1062/1 -> SignalFilter/1062
  Info1/1 -> SignalFilter/1063  "<TrafficState[]>"
  Info1/2 -> SignalFilter/1064  "<ErrorFlag[]>"
  Info1/3 -> Reshape_1065/1  "<CurrentSequence_Fellows[]>"
  Reshape_1065/1 -> SignalFilter/1065
  Info1/4 -> Reshape_1066/1  "<CurrentSegment_Fellows[]>"
  Reshape_1066/1 -> SignalFilter/1066
  Info1/5 -> Reshape_1067/1  "<t_local_Fellows[s]>"
  Reshape_1067/1 -> SignalFilter/1067
  Info1/6 -> Reshape_1068/1  "<CurrentSequence_UserSignals[]>"
  Reshape_1068/1 -> SignalFilter/1068
  Info1/7 -> Reshape_1069/1  "<CurrentSegment_UserSignals[]>"
  Reshape_1069/1 -> SignalFilter/1069
  Info1/8 -> Reshape_1070/1  "<t_local_UserSignals[s]>"
  Reshape_1070/1 -> SignalFilter/1070
  Info1/9 -> SignalFilter/1071  "<CurrentSegment[]>"
  Info1/10 -> SignalFilter/1072  "<t_local[s]>"
  TrafficScheduler/16 -> SignalFilter/1073  "<Dist_Refline_Response[m]>"
  UserSignals_Customized2/1 -> SignalFilter/1074  "<ManeuverSegmentEndTrigger[0|1]>"
  UserSignals_Customized2/2 -> SignalFilter/1075  "<Fellow1_TurnLights>"
  UserSignals_Customized2/3 -> SignalFilter/1076  "<Fellow2_TurnLights>"
  UserSignals_Customized2/4 -> SignalFilter/1077  "<Fellow3_TurnLights>"
  UserSignals_Customized2/5 -> SignalFilter/1078  "<Fellow4_TurnLights>"
  UserSignals_Customized2/6 -> SignalFilter/1079  "<Fellow5_TurnLights>"
  UserSignals_Customized2/7 -> SignalFilter/1080  "<Fellow6_TurnLights>"
  UserSignals_Customized2/8 -> SignalFilter/1081  "<Fellow7_TurnLights>"
  UserSignals_Customized2/9 -> SignalFilter/1082  "<Fellow8_TurnLights>"
  UserSignals_Customized2/10 -> SignalFilter/1083  "<Fellow9_TurnLights>"
  UserSignals_Customized2/11 -> SignalFilter/1084  "<Fellow10_TurnLights>"
  UserSignals_Customized2/12 -> SignalFilter/1085  "<Fellow11_TurnLights>"
  UserSignals_Customized2/13 -> SignalFilter/1086  "<Fellow12_TurnLights>"
  UserSignals_Customized2/14 -> SignalFilter/1087  "<Fellow13_TurnLights>"
  UserSignals_Customized2/15 -> SignalFilter/1088  "<Fellow14_TurnLights>"
  UserSignals_Customized2/16 -> SignalFilter/1089  "<Fellow15_TurnLights>"
  Info2/1 -> SignalFilter/1090  "<FellowParameters_Sfcn_State[]>"
  Info2/2 -> SignalFilter/1091  "<FellowParameters_Data_Valid[0|1]>"
  FellowsGeometry/2 -> Reshape_1092/1  "<Data_Valid_Fellows[0|1]>"
  Reshape_1092/1 -> SignalFilter/1092
  FellowsGeometry/3 -> Reshape_1093/1  "<PosVec_MainPnt_Fellows[x;y;z][m]>"
  Reshape_1093/1 -> SignalFilter/1093
  FellowsGeometry/4 -> Reshape_1094/1  "<Length_Fellows[m]>"
  Reshape_1094/1 -> SignalFilter/1094
  FellowsGeometry/5 -> Reshape_1095/1  "<Width_Fellows[m]>"
  Reshape_1095/1 -> SignalFilter/1095
  FellowsGeometry/6 -> Reshape_1096/1  "<Height_Fellows[m]>"
  Reshape_1096/1 -> SignalFilter/1096
  FellowsGeometry/7 -> Reshape_1097/1  "<Wheel_Radius_Fellows[m]>"
  Reshape_1097/1 -> SignalFilter/1097
  FellowsGeometry/8 -> Reshape_1098/1  "<TrackWidth_Front_Fellows[m]>"
  Reshape_1098/1 -> SignalFilter/1098
  FellowsGeometry/9 -> Reshape_1099/1  "<TrackWidth_Rear_Fellows[m]>"
  Reshape_1099/1 -> SignalFilter/1099
  FellowsGeometry/10 -> Reshape_1100/1  "<WheelBase_Fellows[m]>"
  Reshape_1100/1 -> SignalFilter/1100
  FellowsGeometry/11 -> Reshape_1101/1  "<TrafficObject_Type_Fellows[]>"
  Reshape_1101/1 -> SignalFilter/1101
  TrafficObjects/1 -> SignalFilter/1102  "<TrafficObjectsState[]>"
  TrafficObjects/2 -> DataTypeConversion_1103/1  "<Data_Valid[]>"
  DataTypeConversion_1103/1 -> SignalFilter/1103
  DiscreteObjects/1 -> SignalFilter/1104  "<DiscreteObjectsState[]>"
  DiscreteObjects/2 -> DataTypeConversion_1105/1  "<Data_Valid[]>"
  DataTypeConversion_1105/1 -> SignalFilter/1105
  Sample_Pulse/1 -> DataTypeConversion_1106/1  "<Pulse[0|1]>"
  DataTypeConversion_1106/1 -> SignalFilter/1106
  Sensor_Scheduler/1 -> SignalFilter/1107  "<SensorEnable[0Off|1On]>"
  Sensor_Scheduler/2 -> SignalFilter/1108  "<SensorIdx_Selected[]>"
  Sensor_Scheduler/3 -> SignalFilter/1109  "<Conflict_Flag[0|1]>"
  Sensor_Scheduler/4 -> Reshape_1110/1  "<CylceConflict_Info[]>"
  Reshape_1110/1 -> SignalFilter/1110
  Sensor_Scheduler/5 -> Reshape_1111/1  "<IndexConflict_Info[]>"
  Reshape_1111/1 -> SignalFilter/1111
  Sensor_Scheduler/6 -> Reshape_1112/1  "<SensorSelection_Data[0|1]>"
  Reshape_1112/1 -> SignalFilter/1112
  Sensor_Scheduler/7 -> Reshape_1113/1  "<DelayPulse_SensorOutput[0|1]>"
  Reshape_1113/1 -> SignalFilter/1113
  Parameter/1 -> SignalFilter/1114  "<Sensor_Enable[0Off|1On]>"
  Parameter/2 -> SignalFilter/1115  "<SensorIdx[]>"
  Parameter/3 -> SignalFilter/1116  "<t_Offs_Sensor[s]>"
  Parameter/4 -> SignalFilter/1117  "<t_Cycle_Sensor[s]>"
  Parameter/5 -> SignalFilter/1118  "<t_Delay_SensorOutput[s]>"
  Parameter/6 -> SignalFilter/1119  "<Geometry[]>"
  Parameter/7 -> Reshape_1120/1  "<Pos_Sensor_Apex_CoorSys_V[x;y;z][m]>"
  Reshape_1120/1 -> SignalFilter/1120
  Parameter/8 -> Reshape_1121/1  "<Angle_Orientation_Sensor_CoorSys_V[x;y;z][deg]>"
  Reshape_1121/1 -> SignalFilter/1121
  Parameter/9 -> SignalFilter/1122  "<Length_ScopeZone[m]>"
  Parameter/10 -> SignalFilter/1123  "<Angle_ScopeZone_Horizontal[deg]>"
  Parameter/11 -> SignalFilter/1124  "<Angle_ScopeZone_Vertical[deg]>"
  Parameter/12 -> SignalFilter/1125  "<Length_ScopeZone_Head[m]>"
  Parameter/13 -> SignalFilter/1126  "<Length_BlindZone[m]>"
  Parameter/14 -> SignalFilter/1127  "<Occlusion_Mode[1No_Occlusion|2Basic_3D|3Occlusion_Ratio_3D]>"
  Parameter/15 -> SignalFilter/1128  "<Threshold_Occlusion_Ratio[0_1]>"
  Parameter/16 -> SignalFilter/1129  "<Object_Points_Calculation_Enable[0Off|1On]>"
  Parameter/17 -> SignalFilter/1130  "<Object_Points_Occlusion_Enable[0Off|1On]>"
  SensorIndex/1 -> SignalFilter/1131  "<Idx_Sensor[]>"
  Info3/1 -> Reshape_1132/1  "<Flag_Object_In_Scope[0Out|1In]>"
  Reshape_1132/1 -> SignalFilter/1132
  Info3/2 -> Reshape_1133/1  "<Flag_Sensor_Apex_In_Object[0Out|1In]>"
  Reshape_1133/1 -> SignalFilter/1133
  SensorOutput/1 -> Reshape_1134/1  "<v_Rel_Object[m|s]>"
  Reshape_1134/1 -> SignalFilter/1134
  SensorOutput/2 -> Reshape_1135/1  "<a_Rel_Object[m|s2]>"
  Reshape_1135/1 -> SignalFilter/1135
  SensorOutput/3 -> Reshape_1136/1  "<Dist_Object[m]>"
  Reshape_1136/1 -> SignalFilter/1136
  SensorOutput/4 -> Reshape_1137/1  "<Angle_Hor_Object[deg]>"
  Reshape_1137/1 -> SignalFilter/1137
  SensorOutput/5 -> Reshape_1138/1  "<Angle_Ver_Object[deg]>"
  Reshape_1138/1 -> SignalFilter/1138
  SensorOutput/6 -> Reshape_1139/1  "<Pos_Sensor_Apex_E[x;y;z][m]>"
  Reshape_1139/1 -> SignalFilter/1139
  SensorOutput/7 -> Reshape_1140/1  "<Pos_Object_NearestPnt_E[x;y;z][m]>"
  Reshape_1140/1 -> SignalFilter/1140
  SensorOutput/8 -> Reshape_1141/1  "<Object_Info[-1None|1Fellow|2Static]>"
  Reshape_1141/1 -> SignalFilter/1141
  SensorOutput/9 -> Reshape_1142/1  "<Object_ID[]>"
  Reshape_1142/1 -> SignalFilter/1142
  SensorOutput/10 -> Reshape_1143/1  "<Object_Type[]>"
  Reshape_1143/1 -> SignalFilter/1143
  SensorOutput/11 -> Reshape_1144/1  "<Occlusion_Ratio_Object[-1|0_1]>"
  Reshape_1144/1 -> SignalFilter/1144
  SensorOutput/12 -> Reshape_1145/1  "<Flag_NearestPnt_Occluded[-1|0|1]>"
  Reshape_1145/1 -> SignalFilter/1145
  SensorOutput/13 -> Reshape_1146/1  "<Pos_NearestSurf_Pnt1_CoorSys_S[x;y;z][m]>"
  Reshape_1146/1 -> SignalFilter/1146
  SensorOutput/14 -> Reshape_1147/1  "<Pos_NearestSurf_Pnt2_CoorSys_S[x;y;z][m]>"
  Reshape_1147/1 -> SignalFilter/1147
  SensorOutput/15 -> Reshape_1148/1  "<Pos_NearestSurf_Pnt3_CoorSys_S[x;y;z][m]>"
  Reshape_1148/1 -> SignalFilter/1148
  SensorOutput/16 -> Reshape_1149/1  "<Pos_NearestSurf_Pnt4_CoorSys_S[x;y;z][m]>"
  Reshape_1149/1 -> SignalFilter/1149
  SensorOutput/17 -> Reshape_1150/1  "<NearestSurf_Pnts_Index[]>"
  Reshape_1150/1 -> SignalFilter/1150
  SensorOutput/18 -> Reshape_1151/1  "<NearestSurf_Index[]>"
  Reshape_1151/1 -> SignalFilter/1151
  RadarEffects/1 -> Reshape_1152/1  "<ID[]>"
  Reshape_1152/1 -> SignalFilter/1152
  RadarEffects/2 -> Reshape_1153/1  "<Object_ID[]>"
  Reshape_1153/1 -> SignalFilter/1153
  RadarEffects/3 -> Reshape_1154/1  "<Dist_CoorSys_S[m]>"
  Reshape_1154/1 -> SignalFilter/1154
  RadarEffects/4 -> Reshape_1155/1  "<Angle_Hor_CoorSys_S[deg]>"
  Reshape_1155/1 -> SignalFilter/1155
  RadarEffects/5 -> Reshape_1156/1  "<Pos_ObjectPoint_CoorSys_E[x;y;z][m]>"
  Reshape_1156/1 -> SignalFilter/1156
  CustomPoints/1 -> Reshape_1157/1  "<ID[]>"
  Reshape_1157/1 -> SignalFilter/1157
  CustomPoints/2 -> Reshape_1158/1  "<Object_ID[]>"
  Reshape_1158/1 -> SignalFilter/1158
  CustomPoints/3 -> Reshape_1159/1  "<Dist_CoorSys_S[m]>"
  Reshape_1159/1 -> SignalFilter/1159
  CustomPoints/4 -> Reshape_1160/1  "<Angle_Hor_CoorSys_S[deg]>"
  Reshape_1160/1 -> SignalFilter/1160
  CustomPoints/5 -> Reshape_1161/1  "<Pos_CoorSys_E[x;y;z][m]>"
  Reshape_1161/1 -> SignalFilter/1161
  Parameter1/1 -> SignalFilter/1162  "<Sensor_Enable[0Off|1On]>"
  Parameter1/2 -> SignalFilter/1163  "<SensorIdx[]>"
  Parameter1/3 -> SignalFilter/1164  "<t_Offs_Sensor[s]>"
  Parameter1/4 -> SignalFilter/1165  "<t_Cycle_Sensor[s]>"
  Parameter1/5 -> SignalFilter/1166  "<t_Delay_SensorOutput[s]>"
  Parameter1/6 -> SignalFilter/1167  "<Geometry[]>"
  Parameter1/7 -> Reshape_1168/1  "<Pos_Sensor_Apex_CoorSys_V[x;y;z][m]>"
  Reshape_1168/1 -> SignalFilter/1168
  Parameter1/8 -> Reshape_1169/1  "<Angle_Orientation_Sensor_CoorSys_V[x;y;z][deg]>"
  Reshape_1169/1 -> SignalFilter/1169
  Parameter1/9 -> SignalFilter/1170  "<Length_ScopeZone[m]>"
  Parameter1/10 -> SignalFilter/1171  "<Angle_ScopeZone_Horizontal[deg]>"
  Parameter1/11 -> SignalFilter/1172  "<Angle_ScopeZone_Vertical[deg]>"
  Parameter1/12 -> SignalFilter/1173  "<Length_ScopeZone_Head[m]>"
  Parameter1/13 -> SignalFilter/1174  "<Length_BlindZone[m]>"
  Parameter1/14 -> SignalFilter/1175  "<Occlusion_Mode[1No_Occlusion|2Basic_3D|3Occlusion_Ratio_3D]>"
  Parameter1/15 -> SignalFilter/1176  "<Threshold_Occlusion_Ratio[0_1]>"
  Parameter1/16 -> SignalFilter/1177  "<Object_Points_Calculation_Enable[0Off|1On]>"
  Parameter1/17 -> SignalFilter/1178  "<Object_Points_Occlusion_Enable[0Off|1On]>"
  SensorIndex1/1 -> SignalFilter/1179  "<Idx_Sensor[]>"
  Info4/1 -> Reshape_1180/1  "<Flag_Object_In_Scope[0Out|1In]>"
  Reshape_1180/1 -> SignalFilter/1180
  Info4/2 -> Reshape_1181/1  "<Flag_Sensor_Apex_In_Object[0Out|1In]>"
  Reshape_1181/1 -> SignalFilter/1181
  SensorOutput1/1 -> Reshape_1182/1  "<v_Rel_Object[m|s]>"
  Reshape_1182/1 -> SignalFilter/1182
  SensorOutput1/2 -> Reshape_1183/1  "<a_Rel_Object[m|s2]>"
  Reshape_1183/1 -> SignalFilter/1183
  SensorOutput1/3 -> Reshape_1184/1  "<Dist_Object[m]>"
  Reshape_1184/1 -> SignalFilter/1184
  SensorOutput1/4 -> Reshape_1185/1  "<Angle_Hor_Object[deg]>"
  Reshape_1185/1 -> SignalFilter/1185
  SensorOutput1/5 -> Reshape_1186/1  "<Angle_Ver_Object[deg]>"
  Reshape_1186/1 -> SignalFilter/1186
  SensorOutput1/6 -> Reshape_1187/1  "<Pos_Sensor_Apex_E[x;y;z][m]>"
  Reshape_1187/1 -> SignalFilter/1187
  SensorOutput1/7 -> Reshape_1188/1  "<Pos_Object_NearestPnt_E[x;y;z][m]>"
  Reshape_1188/1 -> SignalFilter/1188
  SensorOutput1/8 -> Reshape_1189/1  "<Object_Info[-1None|1Fellow|2Static]>"
  Reshape_1189/1 -> SignalFilter/1189
  SensorOutput1/9 -> Reshape_1190/1  "<Object_ID[]>"
  Reshape_1190/1 -> SignalFilter/1190
  SensorOutput1/10 -> Reshape_1191/1  "<Object_Type[]>"
  Reshape_1191/1 -> SignalFilter/1191
  SensorOutput1/11 -> Reshape_1192/1  "<Occlusion_Ratio_Object[-1|0_1]>"
  Reshape_1192/1 -> SignalFilter/1192
  SensorOutput1/12 -> Reshape_1193/1  "<Flag_NearestPnt_Occluded[-1|0|1]>"
  Reshape_1193/1 -> SignalFilter/1193
  SensorOutput1/13 -> Reshape_1194/1  "<Pos_NearestSurf_Pnt1_CoorSys_S[x;y;z][m]>"
  Reshape_1194/1 -> SignalFilter/1194
  SensorOutput1/14 -> Reshape_1195/1  "<Pos_NearestSurf_Pnt2_CoorSys_S[x;y;z][m]>"
  Reshape_1195/1 -> SignalFilter/1195
  SensorOutput1/15 -> Reshape_1196/1  "<Pos_NearestSurf_Pnt3_CoorSys_S[x;y;z][m]>"
  Reshape_1196/1 -> SignalFilter/1196
  SensorOutput1/16 -> Reshape_1197/1  "<Pos_NearestSurf_Pnt4_CoorSys_S[x;y;z][m]>"
  Reshape_1197/1 -> SignalFilter/1197
  SensorOutput1/17 -> Reshape_1198/1  "<NearestSurf_Pnts_Index[]>"
  Reshape_1198/1 -> SignalFilter/1198
  SensorOutput1/18 -> Reshape_1199/1  "<NearestSurf_Index[]>"
  Reshape_1199/1 -> SignalFilter/1199
  RadarEffects1/1 -> Reshape_1200/1  "<ID[]>"
  Reshape_1200/1 -> SignalFilter/1200
  RadarEffects1/2 -> Reshape_1201/1  "<Object_ID[]>"
  Reshape_1201/1 -> SignalFilter/1201
  RadarEffects1/3 -> Reshape_1202/1  "<Dist_CoorSys_S[m]>"
  Reshape_1202/1 -> SignalFilter/1202
  RadarEffects1/4 -> Reshape_1203/1  "<Angle_Hor_CoorSys_S[deg]>"
  Reshape_1203/1 -> SignalFilter/1203
  RadarEffects1/5 -> Reshape_1204/1  "<Pos_ObjectPoint_CoorSys_E[x;y;z][m]>"
  Reshape_1204/1 -> SignalFilter/1204
  CustomPoints1/1 -> Reshape_1205/1  "<ID[]>"
  Reshape_1205/1 -> SignalFilter/1205
  CustomPoints1/2 -> Reshape_1206/1  "<Object_ID[]>"
  Reshape_1206/1 -> SignalFilter/1206
  CustomPoints1/3 -> Reshape_1207/1  "<Dist_CoorSys_S[m]>"
  Reshape_1207/1 -> SignalFilter/1207
  CustomPoints1/4 -> Reshape_1208/1  "<Angle_Hor_CoorSys_S[deg]>"
  Reshape_1208/1 -> SignalFilter/1208
  CustomPoints1/5 -> Reshape_1209/1  "<Pos_CoorSys_E[x;y;z][m]>"
  Reshape_1209/1 -> SignalFilter/1209
  Parameter2/1 -> SignalFilter/1210  "<Sensor_Enable[0Off|1On]>"
  Parameter2/2 -> SignalFilter/1211  "<SensorIdx[]>"
  Parameter2/3 -> SignalFilter/1212  "<t_Offs_Sensor[s]>"
  Parameter2/4 -> SignalFilter/1213  "<t_Cycle_Sensor[s]>"
  Parameter2/5 -> SignalFilter/1214  "<t_Delay_SensorOutput[s]>"
  Parameter2/6 -> SignalFilter/1215  "<Geometry[]>"
  Parameter2/7 -> Reshape_1216/1  "<Pos_Sensor_Apex_CoorSys_V[x;y;z][m]>"
  Reshape_1216/1 -> SignalFilter/1216
  Parameter2/8 -> Reshape_1217/1  "<Angle_Orientation_Sensor_CoorSys_V[x;y;z][deg]>"
  Reshape_1217/1 -> SignalFilter/1217
  Parameter2/9 -> SignalFilter/1218  "<Length_ScopeZone[m]>"
  Parameter2/10 -> SignalFilter/1219  "<Angle_ScopeZone_Horizontal[deg]>"
  Parameter2/11 -> SignalFilter/1220  "<Angle_ScopeZone_Vertical[deg]>"
  Parameter2/12 -> SignalFilter/1221  "<Length_ScopeZone_Head[m]>"
  Parameter2/13 -> SignalFilter/1222  "<Length_BlindZone[m]>"
  Parameter2/14 -> SignalFilter/1223  "<Occlusion_Mode[1No_Occlusion|2Basic_3D|3Occlusion_Ratio_3D]>"
  Parameter2/15 -> SignalFilter/1224  "<Threshold_Occlusion_Ratio[0_1]>"
  Parameter2/16 -> SignalFilter/1225  "<Object_Points_Calculation_Enable[0Off|1On]>"
  Parameter2/17 -> SignalFilter/1226  "<Object_Points_Occlusion_Enable[0Off|1On]>"
  SensorIndex2/1 -> SignalFilter/1227  "<Idx_Sensor[]>"
  Info5/1 -> Reshape_1228/1  "<Flag_Object_In_Scope[0Out|1In]>"
  Reshape_1228/1 -> SignalFilter/1228
  Info5/2 -> Reshape_1229/1  "<Flag_Sensor_Apex_In_Object[0Out|1In]>"
  Reshape_1229/1 -> SignalFilter/1229
  SensorOutput2/1 -> Reshape_1230/1  "<v_Rel_Object[m|s]>"
  Reshape_1230/1 -> SignalFilter/1230
  SensorOutput2/2 -> Reshape_1231/1  "<a_Rel_Object[m|s2]>"
  Reshape_1231/1 -> SignalFilter/1231
  SensorOutput2/3 -> Reshape_1232/1  "<Dist_Object[m]>"
  Reshape_1232/1 -> SignalFilter/1232
  SensorOutput2/4 -> Reshape_1233/1  "<Angle_Hor_Object[deg]>"
  Reshape_1233/1 -> SignalFilter/1233
  SensorOutput2/5 -> Reshape_1234/1  "<Angle_Ver_Object[deg]>"
  Reshape_1234/1 -> SignalFilter/1234
  SensorOutput2/6 -> Reshape_1235/1  "<Pos_Sensor_Apex_E[x;y;z][m]>"
  Reshape_1235/1 -> SignalFilter/1235
  SensorOutput2/7 -> Reshape_1236/1  "<Pos_Object_NearestPnt_E[x;y;z][m]>"
  Reshape_1236/1 -> SignalFilter/1236
  SensorOutput2/8 -> Reshape_1237/1  "<Object_Info[-1None|1Fellow|2Static]>"
  Reshape_1237/1 -> SignalFilter/1237
  SensorOutput2/9 -> Reshape_1238/1  "<Object_ID[]>"
  Reshape_1238/1 -> SignalFilter/1238
  SensorOutput2/10 -> Reshape_1239/1  "<Object_Type[]>"
  Reshape_1239/1 -> SignalFilter/1239
  SensorOutput2/11 -> Reshape_1240/1  "<Occlusion_Ratio_Object[-1|0_1]>"
  Reshape_1240/1 -> SignalFilter/1240
  SensorOutput2/12 -> Reshape_1241/1  "<Flag_NearestPnt_Occluded[-1|0|1]>"
  Reshape_1241/1 -> SignalFilter/1241
  SensorOutput2/13 -> Reshape_1242/1  "<Pos_NearestSurf_Pnt1_CoorSys_S[x;y;z][m]>"
  Reshape_1242/1 -> SignalFilter/1242
  SensorOutput2/14 -> Reshape_1243/1  "<Pos_NearestSurf_Pnt2_CoorSys_S[x;y;z][m]>"
  Reshape_1243/1 -> SignalFilter/1243
  SensorOutput2/15 -> Reshape_1244/1  "<Pos_NearestSurf_Pnt3_CoorSys_S[x;y;z][m]>"
  Reshape_1244/1 -> SignalFilter/1244
  SensorOutput2/16 -> Reshape_1245/1  "<Pos_NearestSurf_Pnt4_CoorSys_S[x;y;z][m]>"
  Reshape_1245/1 -> SignalFilter/1245
  SensorOutput2/17 -> Reshape_1246/1  "<NearestSurf_Pnts_Index[]>"
  Reshape_1246/1 -> SignalFilter/1246
  SensorOutput2/18 -> Reshape_1247/1  "<NearestSurf_Index[]>"
  Reshape_1247/1 -> SignalFilter/1247
  RadarEffects2/1 -> Reshape_1248/1  "<ID[]>"
  Reshape_1248/1 -> SignalFilter/1248
  RadarEffects2/2 -> Reshape_1249/1  "<Object_ID[]>"
  Reshape_1249/1 -> SignalFilter/1249
  RadarEffects2/3 -> Reshape_1250/1  "<Dist_CoorSys_S[m]>"
  Reshape_1250/1 -> SignalFilter/1250
  RadarEffects2/4 -> Reshape_1251/1  "<Angle_Hor_CoorSys_S[deg]>"
  Reshape_1251/1 -> SignalFilter/1251
  RadarEffects2/5 -> Reshape_1252/1  "<Pos_ObjectPoint_CoorSys_E[x;y;z][m]>"
  Reshape_1252/1 -> SignalFilter/1252
  CustomPoints2/1 -> Reshape_1253/1  "<ID[]>"
  Reshape_1253/1 -> SignalFilter/1253
  CustomPoints2/2 -> Reshape_1254/1  "<Object_ID[]>"
  Reshape_1254/1 -> SignalFilter/1254
  CustomPoints2/3 -> Reshape_1255/1  "<Dist_CoorSys_S[m]>"
  Reshape_1255/1 -> SignalFilter/1255
  CustomPoints2/4 -> Reshape_1256/1  "<Angle_Hor_CoorSys_S[deg]>"
  Reshape_1256/1 -> SignalFilter/1256
  CustomPoints2/5 -> Reshape_1257/1  "<Pos_CoorSys_E[x;y;z][m]>"
  Reshape_1257/1 -> SignalFilter/1257
  Sample_Pulse1/1 -> DataTypeConversion_1258/1  "<Pulse[0|1]>"
  DataTypeConversion_1258/1 -> SignalFilter/1258
  Sensor_Scheduler1/1 -> SignalFilter/1259  "<SensorEnable[0Off|1On]>"
  Sensor_Scheduler1/2 -> SignalFilter/1260  "<SensorIdx_Selected[]>"
  Sensor_Scheduler1/3 -> SignalFilter/1261  "<Conflict_Flag[0|1]>"
  Sensor_Scheduler1/4 -> Reshape_1262/1  "<CylceConflict_Info[]>"
  Reshape_1262/1 -> SignalFilter/1262
  Sensor_Scheduler1/5 -> Reshape_1263/1  "<IndexConflict_Info[]>"
  Reshape_1263/1 -> SignalFilter/1263
  Sensor_Scheduler1/6 -> Reshape_1264/1  "<SensorSelection_Data[0|1]>"
  Reshape_1264/1 -> SignalFilter/1264
  Sensor_Scheduler1/7 -> Reshape_1265/1  "<DelayPulse_SensorOutput[0|1]>"
  Reshape_1265/1 -> SignalFilter/1265
  Parameters2/1 -> SignalFilter/1266  "<Sensor_Enable[0Off|1On]>"
  Parameters2/2 -> SignalFilter/1267  "<SensorIdx[]>"
  Parameters2/3 -> SignalFilter/1268  "<t_Offs_Sensor[s]>"
  Parameters2/4 -> SignalFilter/1269  "<t_Cycle_Sensor[s]>"
  Parameters2/5 -> SignalFilter/1270  "<t_Delay_SensorOutput[s]>"
  Parameters2/6 -> Reshape_1271/1  "<Pos_Sensor_Apex_CoorSys_V[x;y;z][m]>"
  Reshape_1271/1 -> SignalFilter/1271
  Parameters2/7 -> SignalFilter/1272  "<Angle_z_Orientation_Sensor_CoorSys_V[deg]>"
  Parameters2/8 -> SignalFilter/1273  "<Angle_ScopeZone_Horizontal[deg]>"
  Parameters2/9 -> SignalFilter/1274  "<Length_ScopeZone[m]>"
  Parameters2/10 -> SignalFilter/1275  "<Num_SensorRays_Used[]>"
  Parameters2/11 -> SignalFilter/1276  "<Sensor_Detection_Mode[1Ray|2Sector]>"
  Parameters2/12 -> SignalFilter/1277  "<Object_Detection_Mode[1Object|2Continuous|3All]>"
  SensorIndex3/1 -> SignalFilter/1278  "<Idx_Sensor[]>"
  SensorStatus/1 -> SignalFilter/1279  "<Flag_Object_In_Scope[0Out|1In]>"
  SensorStatus/2 -> SignalFilter/1280  "<Flag_Sensor_Apex_In_Object[0Out|1In]>"
  SensorOutput3/1 -> Reshape_1281/1  "<Angle_Hor_Rel[deg]>"
  Reshape_1281/1 -> SignalFilter/1281
  SensorOutput3/2 -> Reshape_1282/1  "<Object_ID[]>"
  Reshape_1282/1 -> SignalFilter/1282
  SensorOutput3/3 -> Reshape_1283/1  "<Object_Type[]>"
  Reshape_1283/1 -> SignalFilter/1283
  SensorOutput3/4 -> Reshape_1284/1  "<Distance[m]>"
  Reshape_1284/1 -> SignalFilter/1284
  SensorOutput3/5 -> Reshape_1285/1  "<v_Rel[m|s]>"
  Reshape_1285/1 -> SignalFilter/1285
  SensorOutput3/6 -> Reshape_1286/1  "<a_Rel[m|s2]>"
  Reshape_1286/1 -> SignalFilter/1286
  SensorOutput3/7 -> Reshape_1287/1  "<Height_Min[m]>"
  Reshape_1287/1 -> SignalFilter/1287
  SensorOutput3/8 -> Reshape_1288/1  "<Height_Max[m]>"
  Reshape_1288/1 -> SignalFilter/1288
  Info6/1 -> SignalFilter/1289  "<ObjectSensor2D_Sfcn_State[]>"
  Info6/2 -> SignalFilter/1290  "<ObjectSensor2D_Data_Valid[0|1]>"
  Parameters3/1 -> SignalFilter/1291  "<Sensor_Enable[0Off|1On]>"
  Parameters3/2 -> SignalFilter/1292  "<SensorIdx[]>"
  Parameters3/3 -> SignalFilter/1293  "<t_Offs_Sensor[s]>"
  Parameters3/4 -> SignalFilter/1294  "<t_Cycle_Sensor[s]>"
  Parameters3/5 -> SignalFilter/1295  "<t_Delay_SensorOutput[s]>"
  Parameters3/6 -> Reshape_1296/1  "<Pos_Sensor_Apex_CoorSys_V[x;y;z][m]>"
  Reshape_1296/1 -> SignalFilter/1296
  Parameters3/7 -> SignalFilter/1297  "<Angle_z_Orientation_Sensor_CoorSys_V[deg]>"
  Parameters3/8 -> SignalFilter/1298  "<Angle_ScopeZone_Horizontal[deg]>"
  Parameters3/9 -> SignalFilter/1299  "<Length_ScopeZone[m]>"
  Parameters3/10 -> SignalFilter/1300  "<Num_SensorRays_Used[]>"
  Parameters3/11 -> SignalFilter/1301  "<Sensor_Detection_Mode[1Ray|2Sector]>"
  Parameters3/12 -> SignalFilter/1302  "<Object_Detection_Mode[1Object|2Continuous|3All]>"
  SensorIndex4/1 -> SignalFilter/1303  "<Idx_Sensor[]>"
  SensorStatus1/1 -> SignalFilter/1304  "<Flag_Object_In_Scope[0Out|1In]>"
  SensorStatus1/2 -> SignalFilter/1305  "<Flag_Sensor_Apex_In_Object[0Out|1In]>"
  SensorOutput4/1 -> Reshape_1306/1  "<Angle_Hor_Rel[deg]>"
  Reshape_1306/1 -> SignalFilter/1306
  SensorOutput4/2 -> Reshape_1307/1  "<Object_ID[]>"
  Reshape_1307/1 -> SignalFilter/1307
  SensorOutput4/3 -> Reshape_1308/1  "<Object_Type[]>"
  Reshape_1308/1 -> SignalFilter/1308
  SensorOutput4/4 -> Reshape_1309/1  "<Distance[m]>"
  Reshape_1309/1 -> SignalFilter/1309
  SensorOutput4/5 -> Reshape_1310/1  "<v_Rel[m|s]>"
  Reshape_1310/1 -> SignalFilter/1310
  SensorOutput4/6 -> Reshape_1311/1  "<a_Rel[m|s2]>"
  Reshape_1311/1 -> SignalFilter/1311
  SensorOutput4/7 -> Reshape_1312/1  "<Height_Min[m]>"
  Reshape_1312/1 -> SignalFilter/1312
  SensorOutput4/8 -> Reshape_1313/1  "<Height_Max[m]>"
  Reshape_1313/1 -> SignalFilter/1313
  Info7/1 -> SignalFilter/1314  "<ObjectSensor2D_Sfcn_State[]>"
  Info7/2 -> SignalFilter/1315  "<ObjectSensor2D_Data_Valid[0|1]>"
  Parameters4/1 -> SignalFilter/1316  "<Sensor_Enable[0Off|1On]>"
  Parameters4/2 -> SignalFilter/1317  "<SensorIdx[]>"
  Parameters4/3 -> SignalFilter/1318  "<t_Offs_Sensor[s]>"
  Parameters4/4 -> SignalFilter/1319  "<t_Cycle_Sensor[s]>"
  Parameters4/5 -> SignalFilter/1320  "<t_Delay_SensorOutput[s]>"
  Parameters4/6 -> Reshape_1321/1  "<Pos_Sensor_Apex_CoorSys_V[x;y;z][m]>"
  Reshape_1321/1 -> SignalFilter/1321
  Parameters4/7 -> SignalFilter/1322  "<Angle_z_Orientation_Sensor_CoorSys_V[deg]>"
  Parameters4/8 -> SignalFilter/1323  "<Angle_ScopeZone_Horizontal[deg]>"
  Parameters4/9 -> SignalFilter/1324  "<Length_ScopeZone[m]>"
  Parameters4/10 -> SignalFilter/1325  "<Num_SensorRays_Used[]>"
  Parameters4/11 -> SignalFilter/1326  "<Sensor_Detection_Mode[1Ray|2Sector]>"
  Parameters4/12 -> SignalFilter/1327  "<Object_Detection_Mode[1Object|2Continuous|3All]>"
  SensorIndex5/1 -> SignalFilter/1328  "<Idx_Sensor[]>"
  SensorStatus2/1 -> SignalFilter/1329  "<Flag_Object_In_Scope[0Out|1In]>"
  SensorStatus2/2 -> SignalFilter/1330  "<Flag_Sensor_Apex_In_Object[0Out|1In]>"
  SensorOutput5/1 -> Reshape_1331/1  "<Angle_Hor_Rel[deg]>"
  Reshape_1331/1 -> SignalFilter/1331
  SensorOutput5/2 -> Reshape_1332/1  "<Object_ID[]>"
  Reshape_1332/1 -> SignalFilter/1332
  SensorOutput5/3 -> Reshape_1333/1  "<Object_Type[]>"
  Reshape_1333/1 -> SignalFilter/1333
  SensorOutput5/4 -> Reshape_1334/1  "<Distance[m]>"
  Reshape_1334/1 -> SignalFilter/1334
  SensorOutput5/5 -> Reshape_1335/1  "<v_Rel[m|s]>"
  Reshape_1335/1 -> SignalFilter/1335
  SensorOutput5/6 -> Reshape_1336/1  "<a_Rel[m|s2]>"
  Reshape_1336/1 -> SignalFilter/1336
  SensorOutput5/7 -> Reshape_1337/1  "<Height_Min[m]>"
  Reshape_1337/1 -> SignalFilter/1337
  SensorOutput5/8 -> Reshape_1338/1  "<Height_Max[m]>"
  Reshape_1338/1 -> SignalFilter/1338
  Info8/1 -> SignalFilter/1339  "<ObjectSensor2D_Sfcn_State[]>"
  Info8/2 -> SignalFilter/1340  "<ObjectSensor2D_Data_Valid[0|1]>"
  Parameters5/1 -> SignalFilter/1341  "<Sensor_Enable[0Off|1On]>"
  Parameters5/2 -> SignalFilter/1342  "<SensorIdx[]>"
  Parameters5/3 -> SignalFilter/1343  "<t_Offs_Sensor[s]>"
  Parameters5/4 -> SignalFilter/1344  "<t_Cycle_Sensor[s]>"
  Parameters5/5 -> SignalFilter/1345  "<t_Delay_SensorOutput[s]>"
  Parameters5/6 -> Reshape_1346/1  "<Pos_Sensor_Apex_CoorSys_V[x;y;z][m]>"
  Reshape_1346/1 -> SignalFilter/1346
  Parameters5/7 -> SignalFilter/1347  "<Angle_z_Orientation_Sensor_CoorSys_V[deg]>"
  Parameters5/8 -> SignalFilter/1348  "<Angle_ScopeZone_Horizontal[deg]>"
  Parameters5/9 -> SignalFilter/1349  "<Length_ScopeZone[m]>"
  Parameters5/10 -> SignalFilter/1350  "<Num_SensorRays_Used[]>"
  Parameters5/11 -> SignalFilter/1351  "<Sensor_Detection_Mode[1Ray|2Sector]>"
  Parameters5/12 -> SignalFilter/1352  "<Object_Detection_Mode[1Object|2Continuous|3All]>"
  SensorIndex6/1 -> SignalFilter/1353  "<Idx_Sensor[]>"
  SensorStatus3/1 -> SignalFilter/1354  "<Flag_Object_In_Scope[0Out|1In]>"
  SensorStatus3/2 -> SignalFilter/1355  "<Flag_Sensor_Apex_In_Object[0Out|1In]>"
  SensorOutput6/1 -> Reshape_1356/1  "<Angle_Hor_Rel[deg]>"
  Reshape_1356/1 -> SignalFilter/1356
  SensorOutput6/2 -> Reshape_1357/1  "<Object_ID[]>"
  Reshape_1357/1 -> SignalFilter/1357
  SensorOutput6/3 -> Reshape_1358/1  "<Object_Type[]>"
  Reshape_1358/1 -> SignalFilter/1358
  SensorOutput6/4 -> Reshape_1359/1  "<Distance[m]>"
  Reshape_1359/1 -> SignalFilter/1359
  SensorOutput6/5 -> Reshape_1360/1  "<v_Rel[m|s]>"
  Reshape_1360/1 -> SignalFilter/1360
  SensorOutput6/6 -> Reshape_1361/1  "<a_Rel[m|s2]>"
  Reshape_1361/1 -> SignalFilter/1361
  SensorOutput6/7 -> Reshape_1362/1  "<Height_Min[m]>"
  Reshape_1362/1 -> SignalFilter/1362
  SensorOutput6/8 -> Reshape_1363/1  "<Height_Max[m]>"
  Reshape_1363/1 -> SignalFilter/1363
  Info9/1 -> SignalFilter/1364  "<ObjectSensor2D_Sfcn_State[]>"
  Info9/2 -> SignalFilter/1365  "<ObjectSensor2D_Data_Valid[0|1]>"
  Parameters6/1 -> SignalFilter/1366  "<Sensor_Enable[0Off|1On]>"
  Parameters6/2 -> SignalFilter/1367  "<SensorIdx[]>"
  Parameters6/3 -> SignalFilter/1368  "<t_Offs_Sensor[s]>"
  Parameters6/4 -> SignalFilter/1369  "<t_Cycle_Sensor[s]>"
  Parameters6/5 -> SignalFilter/1370  "<t_Delay_SensorOutput[s]>"
  Parameters6/6 -> Reshape_1371/1  "<Pos_Sensor_Apex_CoorSys_V[x;y;z][m]>"
  Reshape_1371/1 -> SignalFilter/1371
  Parameters6/7 -> SignalFilter/1372  "<Angle_z_Orientation_Sensor_CoorSys_V[deg]>"
  Parameters6/8 -> SignalFilter/1373  "<Angle_ScopeZone_Horizontal[deg]>"
  Parameters6/9 -> SignalFilter/1374  "<Length_ScopeZone[m]>"
  Parameters6/10 -> SignalFilter/1375  "<Num_SensorRays_Used[]>"
  Parameters6/11 -> SignalFilter/1376  "<Sensor_Detection_Mode[1Ray|2Sector]>"
  Parameters6/12 -> SignalFilter/1377  "<Object_Detection_Mode[1Object|2Continuous|3All]>"
  SensorIndex7/1 -> SignalFilter/1378  "<Idx_Sensor[]>"
  SensorStatus4/1 -> SignalFilter/1379  "<Flag_Object_In_Scope[0Out|1In]>"
  SensorStatus4/2 -> SignalFilter/1380  "<Flag_Sensor_Apex_In_Object[0Out|1In]>"
  SensorOutput7/1 -> Reshape_1381/1  "<Angle_Hor_Rel[deg]>"
  Reshape_1381/1 -> SignalFilter/1381
  SensorOutput7/2 -> Reshape_1382/1  "<Object_ID[]>"
  Reshape_1382/1 -> SignalFilter/1382
  SensorOutput7/3 -> Reshape_1383/1  "<Object_Type[]>"
  Reshape_1383/1 -> SignalFilter/1383
  SensorOutput7/4 -> Reshape_1384/1  "<Distance[m]>"
  Reshape_1384/1 -> SignalFilter/1384
  SensorOutput7/5 -> Reshape_1385/1  "<v_Rel[m|s]>"
  Reshape_1385/1 -> SignalFilter/1385
  SensorOutput7/6 -> Reshape_1386/1  "<a_Rel[m|s2]>"
  Reshape_1386/1 -> SignalFilter/1386
  SensorOutput7/7 -> Reshape_1387/1  "<Height_Min[m]>"
  Reshape_1387/1 -> SignalFilter/1387
  SensorOutput7/8 -> Reshape_1388/1  "<Height_Max[m]>"
  Reshape_1388/1 -> SignalFilter/1388
  Info10/1 -> SignalFilter/1389  "<ObjectSensor2D_Sfcn_State[]>"
  Info10/2 -> SignalFilter/1390  "<ObjectSensor2D_Data_Valid[0|1]>"
  Parameters7/1 -> SignalFilter/1391  "<Sensor_Enable[0Off|1On]>"
  Parameters7/2 -> SignalFilter/1392  "<SensorIdx[]>"
  Parameters7/3 -> SignalFilter/1393  "<t_Offs_Sensor[s]>"
  Parameters7/4 -> SignalFilter/1394  "<t_Cycle_Sensor[s]>"
  Parameters7/5 -> SignalFilter/1395  "<t_Delay_SensorOutput[s]>"
  Parameters7/6 -> Reshape_1396/1  "<Pos_Sensor_Apex_CoorSys_V[x;y;z][m]>"
  Reshape_1396/1 -> SignalFilter/1396
  Parameters7/7 -> SignalFilter/1397  "<Angle_z_Orientation_Sensor_CoorSys_V[deg]>"
  Parameters7/8 -> SignalFilter/1398  "<Angle_ScopeZone_Horizontal[deg]>"
  Parameters7/9 -> SignalFilter/1399  "<Length_ScopeZone[m]>"
  Parameters7/10 -> SignalFilter/1400  "<Num_SensorRays_Used[]>"
  Parameters7/11 -> SignalFilter/1401  "<Sensor_Detection_Mode[1Ray|2Sector]>"
  Parameters7/12 -> SignalFilter/1402  "<Object_Detection_Mode[1Object|2Continuous|3All]>"
  SensorIndex8/1 -> SignalFilter/1403  "<Idx_Sensor[]>"
  SensorStatus5/1 -> SignalFilter/1404  "<Flag_Object_In_Scope[0Out|1In]>"
  SensorStatus5/2 -> SignalFilter/1405  "<Flag_Sensor_Apex_In_Object[0Out|1In]>"
  SensorOutput8/1 -> Reshape_1406/1  "<Angle_Hor_Rel[deg]>"
  Reshape_1406/1 -> SignalFilter/1406
  SensorOutput8/2 -> Reshape_1407/1  "<Object_ID[]>"
  Reshape_1407/1 -> SignalFilter/1407
  SensorOutput8/3 -> Reshape_1408/1  "<Object_Type[]>"
  Reshape_1408/1 -> SignalFilter/1408
  SensorOutput8/4 -> Reshape_1409/1  "<Distance[m]>"
  Reshape_1409/1 -> SignalFilter/1409
  SensorOutput8/5 -> Reshape_1410/1  "<v_Rel[m|s]>"
  Reshape_1410/1 -> SignalFilter/1410
  SensorOutput8/6 -> Reshape_1411/1  "<a_Rel[m|s2]>"
  Reshape_1411/1 -> SignalFilter/1411
  SensorOutput8/7 -> Reshape_1412/1  "<Height_Min[m]>"
  Reshape_1412/1 -> SignalFilter/1412
  SensorOutput8/8 -> Reshape_1413/1  "<Height_Max[m]>"
  Reshape_1413/1 -> SignalFilter/1413
  Info11/1 -> SignalFilter/1414  "<ObjectSensor2D_Sfcn_State[]>"
  Info11/2 -> SignalFilter/1415  "<ObjectSensor2D_Data_Valid[0|1]>"
  Parameters8/1 -> SignalFilter/1416  "<Sensor_Enable[0Off|1On]>"
  Parameters8/2 -> SignalFilter/1417  "<SensorIdx[]>"
  Parameters8/3 -> SignalFilter/1418  "<t_Offs_Sensor[s]>"
  Parameters8/4 -> SignalFilter/1419  "<t_Cycle_Sensor[s]>"
  Parameters8/5 -> SignalFilter/1420  "<t_Delay_SensorOutput[s]>"
  Parameters8/6 -> Reshape_1421/1  "<Pos_Sensor_Apex_CoorSys_V[x;y;z][m]>"
  Reshape_1421/1 -> SignalFilter/1421
  Parameters8/7 -> SignalFilter/1422  "<Angle_z_Orientation_Sensor_CoorSys_V[deg]>"
  Parameters8/8 -> SignalFilter/1423  "<Angle_ScopeZone_Horizontal[deg]>"
  Parameters8/9 -> SignalFilter/1424  "<Length_ScopeZone[m]>"
  Parameters8/10 -> SignalFilter/1425  "<Num_SensorRays_Used[]>"
  Parameters8/11 -> SignalFilter/1426  "<Sensor_Detection_Mode[1Ray|2Sector]>"
  Parameters8/12 -> SignalFilter/1427  "<Object_Detection_Mode[1Object|2Continuous|3All]>"
  SensorIndex9/1 -> SignalFilter/1428  "<Idx_Sensor[]>"
  SensorStatus6/1 -> SignalFilter/1429  "<Flag_Object_In_Scope[0Out|1In]>"
  SensorStatus6/2 -> SignalFilter/1430  "<Flag_Sensor_Apex_In_Object[0Out|1In]>"
  SensorOutput9/1 -> Reshape_1431/1  "<Angle_Hor_Rel[deg]>"
  Reshape_1431/1 -> SignalFilter/1431
  SensorOutput9/2 -> Reshape_1432/1  "<Object_ID[]>"
  Reshape_1432/1 -> SignalFilter/1432
  SensorOutput9/3 -> Reshape_1433/1  "<Object_Type[]>"
  Reshape_1433/1 -> SignalFilter/1433
  SensorOutput9/4 -> Reshape_1434/1  "<Distance[m]>"
  Reshape_1434/1 -> SignalFilter/1434
  SensorOutput9/5 -> Reshape_1435/1  "<v_Rel[m|s]>"
  Reshape_1435/1 -> SignalFilter/1435
  SensorOutput9/6 -> Reshape_1436/1  "<a_Rel[m|s2]>"
  Reshape_1436/1 -> SignalFilter/1436
  SensorOutput9/7 -> Reshape_1437/1  "<Height_Min[m]>"
  Reshape_1437/1 -> SignalFilter/1437
  SensorOutput9/8 -> Reshape_1438/1  "<Height_Max[m]>"
  Reshape_1438/1 -> SignalFilter/1438
  Info12/1 -> SignalFilter/1439  "<ObjectSensor2D_Sfcn_State[]>"
  Info12/2 -> SignalFilter/1440  "<ObjectSensor2D_Data_Valid[0|1]>"
  Info13/1 -> SignalFilter/1441  "<TrafficSignSensor_Dyn_Sfcn_State[]>"
  Info13/2 -> SignalFilter/1442  "<TrafficSignSensor_Dyn_Data_Valid[0|1]>"
  SensorOutput[]/1 -> Reshape_1443/1  "<Traffic_Sign_Valid[0|1]>"
  Reshape_1443/1 -> SignalFilter/1443
  SensorOutput[]/2 -> Reshape_1444/1  "<TrafficObject_ID[]>"
  Reshape_1444/1 -> SignalFilter/1444
  SensorOutput[]/3 -> Reshape_1445/1  "<TrafficObject_Type[]>"
  Reshape_1445/1 -> SignalFilter/1445
  SensorOutput[]/4 -> Reshape_1446/1  "<Pos_CoorSys_E[x;y;z][m]>"
  Reshape_1446/1 -> SignalFilter/1446
  SensorOutput[]/5 -> Reshape_1447/1  "<Angle_CoorSys_E[x;y;z][deg]>"
  Reshape_1447/1 -> SignalFilter/1447
  SensorOutput[]/6 -> Reshape_1448/1  "<Pos_CoorSys_S[x;y;z][m]>"
  Reshape_1448/1 -> SignalFilter/1448
  SensorOutput[]/7 -> Reshape_1449/1  "<Angle_Hor_Rel[deg]>"
  Reshape_1449/1 -> SignalFilter/1449
  SensorOutput[]/8 -> Reshape_1450/1  "<Angle_Ver_Rel[deg]>"
  Reshape_1450/1 -> SignalFilter/1450
  SensorOutput[]/9 -> Reshape_1451/1  "<Angle_Sign_Orientation_Rel[deg]>"
  Reshape_1451/1 -> SignalFilter/1451
  SensorOutput[]/10 -> Reshape_1452/1  "<Distance[m]>"
  Reshape_1452/1 -> SignalFilter/1452
  SensorOutput[]/11 -> Reshape_1453/1  "<Traffic_Sign_Type[]>"
  Reshape_1453/1 -> SignalFilter/1453
  SensorOutput[]/12 -> Reshape_1454/1  "<Traffic_Sign_Subtype[]>"
  Reshape_1454/1 -> SignalFilter/1454
  SensorOutput[]/13 -> Reshape_1455/1  "<Traffic_Sign_Value[]>"
  Reshape_1455/1 -> SignalFilter/1455
  SensorOutput[]/14 -> Reshape_1456/1  "<Traffic_Sign_Country[]>"
  Reshape_1456/1 -> SignalFilter/1456
  SensorOutput[]/15 -> Reshape_1457/1  "<Traffic_Sign_Visibility[0_100]>"
  Reshape_1457/1 -> SignalFilter/1457
  SensorOutput[]/16 -> Reshape_1458/1  "<Traffic_Sign_Lanes[]>"
  Reshape_1458/1 -> SignalFilter/1458
  SensorOutput[]/17 -> Reshape_1459/1  "<Object_Stream_ID[]>"
  Reshape_1459/1 -> SignalFilter/1459
  SensorOutput[]/18 -> Reshape_1460/1  "<Object_State[]>"
  Reshape_1460/1 -> SignalFilter/1460
  SensorOutput[]/19 -> Reshape_1461/1  "<Parent_Object_ID[]>"
  Reshape_1461/1 -> SignalFilter/1461
  SensorOutput[]/20 -> Reshape_1462/1  "<Network_Item_Type[0Junction|1Road]>"
  Reshape_1462/1 -> SignalFilter/1462
  SensorOutput[]/21 -> Reshape_1463/1  "<Network_Item_ID[]>"
  Reshape_1463/1 -> SignalFilter/1463
  Parameters9/1 -> SignalFilter/1464  "<Sensor_Enable[0Off|1On]>"
  Parameters9/2 -> Reshape_1465/1  "<Pos_Sensor_Apex_CoorSys_V[x;y;z][m]>"
  Reshape_1465/1 -> SignalFilter/1465
  Parameters9/3 -> Reshape_1466/1  "<Angle_Orientation_Sensor_CoorSys_V[x;y;z][deg]>"
  Reshape_1466/1 -> SignalFilter/1466
  Parameters9/4 -> SignalFilter/1467  "<Length_ScopeZone[m]>"
  Parameters9/5 -> SignalFilter/1468  "<Angle_ScopeZone_Horizontal[deg]>"
  Parameters9/6 -> SignalFilter/1469  "<Angle_ScopeZone_Vertical[deg]>"
  Parameters9/7 -> SignalFilter/1470  "<Angle_Sign_Orientation_Max[deg]>"
  Info14/1 -> SignalFilter/1471  "<CustomSensor_ScopezoneSfcn_State[]>"
  Info14/2 -> SignalFilter/1472  "<CustomSensor_OutputSfcn_State[]>"
  Info14/3 -> SignalFilter/1473  "<CustomSensor_Data_Valid[0|1]>"
  Object1/1 -> SignalFilter/1474  "<Object_Valid[0|1]>"
  Object1/2 -> SignalFilter/1475  "<Object_ID[]>"
  Object1/3 -> SignalFilter/1476  "<Object_Type[]>"
  Object1/4 -> SignalFilter/1477  "<Pos_x_CoorSys_S[m]>"
  Object1/5 -> SignalFilter/1478  "<Pos_y_CoorSys_S[m]>"
  Object1/6 -> SignalFilter/1479  "<Pos_z_CoorSys_S[m]>"
  Object1/7 -> SignalFilter/1480  "<Angle_Hor_Rel[deg]>"
  Object1/8 -> SignalFilter/1481  "<Angle_Ver_Rel[deg]>"
  Object1/9 -> SignalFilter/1482  "<Distance[m]>"
  Object1/10 -> SignalFilter/1483  "<Network_Item_Type[0Junction|1Road]>"
  Object1/11 -> SignalFilter/1484  "<Network_Item_ID[]>"
  Object1/12 -> SignalFilter/1485  "<Parent_Object_ID[]>"
  Object1/13 -> Reshape_1486/1  "<CustomValues[]>"
  Reshape_1486/1 -> SignalFilter/1486
  Object2/1 -> SignalFilter/1487  "<Object_Valid[0|1]>"
  Object2/2 -> SignalFilter/1488  "<Object_ID[]>"
  Object2/3 -> SignalFilter/1489  "<Object_Type[]>"
  Object2/4 -> SignalFilter/1490  "<Pos_x_CoorSys_S[m]>"
  Object2/5 -> SignalFilter/1491  "<Pos_y_CoorSys_S[m]>"
  Object2/6 -> SignalFilter/1492  "<Pos_z_CoorSys_S[m]>"
  Object2/7 -> SignalFilter/1493  "<Angle_Hor_Rel[deg]>"
  Object2/8 -> SignalFilter/1494  "<Angle_Ver_Rel[deg]>"
  Object2/9 -> SignalFilter/1495  "<Distance[m]>"
  Object2/10 -> SignalFilter/1496  "<Network_Item_Type[0Junction|1Road]>"
  Object2/11 -> SignalFilter/1497  "<Network_Item_ID[]>"
  Object2/12 -> SignalFilter/1498  "<Parent_Object_ID[]>"
  Object2/13 -> Reshape_1499/1  "<CustomValues[]>"
  Reshape_1499/1 -> SignalFilter/1499
  Object3/1 -> SignalFilter/1500  "<Object_Valid[0|1]>"
  Object3/2 -> SignalFilter/1501  "<Object_ID[]>"
  Object3/3 -> SignalFilter/1502  "<Object_Type[]>"
  Object3/4 -> SignalFilter/1503  "<Pos_x_CoorSys_S[m]>"
  Object3/5 -> SignalFilter/1504  "<Pos_y_CoorSys_S[m]>"
  Object3/6 -> SignalFilter/1505  "<Pos_z_CoorSys_S[m]>"
  Object3/7 -> SignalFilter/1506  "<Angle_Hor_Rel[deg]>"
  Object3/8 -> SignalFilter/1507  "<Angle_Ver_Rel[deg]>"
  Object3/9 -> SignalFilter/1508  "<Distance[m]>"
  Object3/10 -> SignalFilter/1509  "<Network_Item_Type[0Junction|1Road]>"
  Object3/11 -> SignalFilter/1510  "<Network_Item_ID[]>"
  Object3/12 -> SignalFilter/1511  "<Parent_Object_ID[]>"
  Object3/13 -> Reshape_1512/1  "<CustomValues[]>"
  Reshape_1512/1 -> SignalFilter/1512
  Object4/1 -> SignalFilter/1513  "<Object_Valid[0|1]>"
  Object4/2 -> SignalFilter/1514  "<Object_ID[]>"
  Object4/3 -> SignalFilter/1515  "<Object_Type[]>"
  Object4/4 -> SignalFilter/1516  "<Pos_x_CoorSys_S[m]>"
  Object4/5 -> SignalFilter/1517  "<Pos_y_CoorSys_S[m]>"
  Object4/6 -> SignalFilter/1518  "<Pos_z_CoorSys_S[m]>"
  Object4/7 -> SignalFilter/1519  "<Angle_Hor_Rel[deg]>"
  Object4/8 -> SignalFilter/1520  "<Angle_Ver_Rel[deg]>"
  Object4/9 -> SignalFilter/1521  "<Distance[m]>"
  Object4/10 -> SignalFilter/1522  "<Network_Item_Type[0Junction|1Road]>"
  Object4/11 -> SignalFilter/1523  "<Network_Item_ID[]>"
  Object4/12 -> SignalFilter/1524  "<Parent_Object_ID[]>"
  Object4/13 -> Reshape_1525/1  "<CustomValues[]>"
  Reshape_1525/1 -> SignalFilter/1525
  Object5/1 -> SignalFilter/1526  "<Object_Valid[0|1]>"
  Object5/2 -> SignalFilter/1527  "<Object_ID[]>"
  Object5/3 -> SignalFilter/1528  "<Object_Type[]>"
  Object5/4 -> SignalFilter/1529  "<Pos_x_CoorSys_S[m]>"
  Object5/5 -> SignalFilter/1530  "<Pos_y_CoorSys_S[m]>"
  Object5/6 -> SignalFilter/1531  "<Pos_z_CoorSys_S[m]>"
  Object5/7 -> SignalFilter/1532  "<Angle_Hor_Rel[deg]>"
  Object5/8 -> SignalFilter/1533  "<Angle_Ver_Rel[deg]>"
  Object5/9 -> SignalFilter/1534  "<Distance[m]>"
  Object5/10 -> SignalFilter/1535  "<Network_Item_Type[0Junction|1Road]>"
  Object5/11 -> SignalFilter/1536  "<Network_Item_ID[]>"
  Object5/12 -> SignalFilter/1537  "<Parent_Object_ID[]>"
  Object5/13 -> Reshape_1538/1  "<CustomValues[]>"
  Reshape_1538/1 -> SignalFilter/1538
  Parameters10/1 -> SignalFilter/1539  "<Sensor_Enable[0Off|1On]>"
  Parameters10/2 -> Reshape_1540/1  "<Pos_Sensor_Apex_CoorSys_V[x;y;z][m]>"
  Reshape_1540/1 -> SignalFilter/1540
  Parameters10/3 -> Reshape_1541/1  "<Angle_Orientation_Sensor_CoorSys_V[x;y;z][deg]>"
  Reshape_1541/1 -> SignalFilter/1541
  Parameters10/4 -> SignalFilter/1542  "<Length_ScopeZone[m]>"
  Parameters10/5 -> SignalFilter/1543  "<Angle_ScopeZone_Horizontal[deg]>"
  Parameters10/6 -> SignalFilter/1544  "<Angle_ScopeZone_Vertical[deg]>"
  Info15/1 -> Reshape_1545/1  "<LineSensor_Data_Outport[]>"
  Reshape_1545/1 -> DataTypeConversion_1545/1
  DataTypeConversion_1545/1 -> SignalFilter/1545
  Info15/2 -> SignalFilter/1546  "<LineSensor_Data_Outport_Version[]>"
  Info15/3 -> SignalFilter/1547  "<LineSensor_Data_Valid[0|1|2]>"
  Info15/4 -> SignalFilter/1548  "<Num_Pnts_Detected_Road_Lanes[]>"
  Info15/5 -> SignalFilter/1549  "<Num_Pnts_Detected_Road_Shape_Lines[]>"
  Info15/6 -> SignalFilter/1550  "<Num_Pnts_Detected_Road_Shape_ContObj[]>"
  Info15/7 -> SignalFilter/1551  "<Num_Pnts_Detected_Junction_Borders[]>"
  Info15/8 -> SignalFilter/1552  "<Num_Pnts_Detected_Junction_Shape_Lines[]>"
  Info15/9 -> SignalFilter/1553  "<Num_Pnts_Detected_Junction_Shape_ContObj[]>"
  Pos_Road_Lane_Animation_CoorSys_E/1 -> Reshape_1554/1  "<Pos_x_Road_Lane_Animation_CoorSys_E>"
  Reshape_1554/1 -> SignalFilter/1554
  Pos_Road_Lane_Animation_CoorSys_E/2 -> Reshape_1555/1  "<Pos_y_Road_Lane_Animation_CoorSys_E>"
  Reshape_1555/1 -> SignalFilter/1555
  Pos_Road_Lane_Animation_CoorSys_E/3 -> Reshape_1556/1  "<Pos_z_Road_Lane_Animation_CoorSys_E>"
  Reshape_1556/1 -> SignalFilter/1556
  Pos_Road_Shape_Line_Animation_CoorSys_E/1 -> Reshape_1557/1  "<Pos_x_Road_Shape_Line_Animation_CoorSys_E>"
  Reshape_1557/1 -> SignalFilter/1557
  Pos_Road_Shape_Line_Animation_CoorSys_E/2 -> Reshape_1558/1  "<Pos_y_Road_Shape_Line_Animation_CoorSys_E>"
  Reshape_1558/1 -> SignalFilter/1558
  Pos_Road_Shape_Line_Animation_CoorSys_E/3 -> Reshape_1559/1  "<Pos_z_Road_Shape_Line_Animation_CoorSys_E>"
  Reshape_1559/1 -> SignalFilter/1559
  Pos_Road_Shape_ContObj_Animation_CoorSys_E/1 -> Reshape_1560/1  "<Pos_x_Road_Shape_ContObj_Animation_CoorSys_E>"
  Reshape_1560/1 -> SignalFilter/1560
  Pos_Road_Shape_ContObj_Animation_CoorSys_E/2 -> Reshape_1561/1  "<Pos_y_Road_Shape_ContObj_Animation_CoorSys_E>"
  Reshape_1561/1 -> SignalFilter/1561
  Pos_Road_Shape_ContObj_Animation_CoorSys_E/3 -> Reshape_1562/1  "<Pos_z_Road_Shape_ContObj_Animation_CoorSys_E>"
  Reshape_1562/1 -> SignalFilter/1562
  Pos_Junction_Border_Animation_CoorSys_E/1 -> Reshape_1563/1  "<Pos_x_Junction_Border_Animation_CoorSys_E>"
  Reshape_1563/1 -> SignalFilter/1563
  Pos_Junction_Border_Animation_CoorSys_E/2 -> Reshape_1564/1  "<Pos_y_Junction_Border_Animation_CoorSys_E>"
  Reshape_1564/1 -> SignalFilter/1564
  Pos_Junction_Border_Animation_CoorSys_E/3 -> Reshape_1565/1  "<Pos_z_Junction_Border_Animation_CoorSys_E>"
  Reshape_1565/1 -> SignalFilter/1565
  Pos_Junction_Shape_Line_Animation_CoorSys_E/1 -> Reshape_1566/1  "<Pos_x_Junction_Shape_Line_Animation_CoorSys_E>"
  Reshape_1566/1 -> SignalFilter/1566
  Pos_Junction_Shape_Line_Animation_CoorSys_E/2 -> Reshape_1567/1  "<Pos_y_Junction_Shape_Line_Animation_CoorSys_E>"
  Reshape_1567/1 -> SignalFilter/1567
  Pos_Junction_Shape_Line_Animation_CoorSys_E/3 -> Reshape_1568/1  "<Pos_z_Junction_Shape_Line_Animation_CoorSys_E>"
  Reshape_1568/1 -> SignalFilter/1568
  Pos_Junction_Shape_ContObj_Animation_CoorSys_E/1 -> Reshape_1569/1  "<Pos_x_Junction_Shape_ContObj_Animation_CoorSys_E>"
  Reshape_1569/1 -> SignalFilter/1569
  Pos_Junction_Shape_ContObj_Animation_CoorSys_E/2 -> Reshape_1570/1  "<Pos_y_Junction_Shape_ContObj_Animation_CoorSys_E>"
  Reshape_1570/1 -> SignalFilter/1570
  Pos_Junction_Shape_ContObj_Animation_CoorSys_E/3 -> Reshape_1571/1  "<Pos_z_Junction_Shape_ContObj_Animation_CoorSys_E>"
  Reshape_1571/1 -> SignalFilter/1571
  Line_Sensor_1/8 -> SignalFilter/1572  "<Dummy_SensorOutput>"
  Info16/1 -> SignalFilter/1573  "<Sfunc_State[]>"
  Info16/2 -> SignalFilter/1574  "<Data_Valid[0|1]>"
  SensorOutput11/1 -> SignalFilter/1575  "<Collision_Flag[0NoCollision|1Collision]>"
  SensorOutput11/2 -> SignalFilter/1576  "<Collision_Flag_Held[0NoCollision|1Collision]>"
  SensorOutput11/3 -> Reshape_1577/1  "<Object_ID[]>"
  Reshape_1577/1 -> SignalFilter/1577
  SensorOutput11/4 -> Reshape_1578/1  "<Time_Collision[s]>"
  Reshape_1578/1 -> SignalFilter/1578
  SensorOutput11/5 -> Reshape_1579/1  "<Pos_Collision_Point[x;y][m]>"
  Reshape_1579/1 -> SignalFilter/1579
  SensorOutput11/6 -> Reshape_1580/1  "<v_Collision_CoG_Vehicle[x;y][m|s]>"
  Reshape_1580/1 -> SignalFilter/1580
  SensorOutput11/7 -> Reshape_1581/1  "<v_Collision_CoG_Vehicle_Total[m|s]>"
  Reshape_1581/1 -> SignalFilter/1581
  SensorOutput11/8 -> Reshape_1582/1  "<v_Rel_Collision_Point[x;y][m|s]>"
  Reshape_1582/1 -> SignalFilter/1582
  SensorOutput11/9 -> Reshape_1583/1  "<v_Rel_Collision_Point_Total[m|s]>"
  Reshape_1583/1 -> SignalFilter/1583
  Sensors_Common/1 -> SignalFilter/1584  "<Enable_SensorScheduling[0Off|1On]>"
  SignalFilter/1 -> SignalFilterGain/1
  SignalFilterGain/1 -> MDLD_DATA_CAPTURE/1
